simulink model "ModeStatAndRsp"  (R2018b)
settings: Solver=FixedStepDiscrete  StartTime=0.0  StopTime=10.0  FixedStep=0.01  RelTol=1e-3
undefined symbols (not defined in the file): c_RecvL, c_RecvLR, c_RecvR, IfVeSMSeStNumConfig, KeSMSbMdChime2Enable_Val, KeSMSbSRSPosNumConfig_Val, KeSMSuChmReqDurnTm_Val, KeSMSuChmReqIntlTm_Val, KeSMSuRspStatHldTm_Val, MdRspLocal1, MdTp1, ModeNum, PowerMode1, SrcReqTp1, srsconvert
libraries: RspLib x47, simulink x1
(part 1 of 8)
settings Model: ModifiedComment=sn2xws -- Mon May 30 15:02:40 2022 -- Version 1.7.1  Creator=Huanglu  LastModifiedBy=sn2xws
settings Model: ModifiedHistory=|
  | sn2xws -- Fri Dec 10 13:33:55 2021 -- Version 1.7.1
  | Vescom 7.0增加标定：KeSMSbMdChime2Enable
  | 
  | sn2xws -- Wed Oct 20 14:19:17 2021 -- Version 1.5.2
  | Bug 194428
  | StPassCmprtMd_RfCtrl_Sw_RclRspStat反馈增加新模式5个
  | sn2xws -- Wed Oct 20 14:19:17 2021 -- Version 1.5.1
  | bug 188541
  | 23.46数据库修改引起的增加模式5个
  | sn2xws -- Wed Oct 20 11:08:15 2021 -- Version 1.3.5
  | 4sbsy逻辑修改
  | 
  | sn2xws -- Thu Sep 23 09:51:03 2021 -- Version 1.3.4
  | 
  | sn2xws -- Thu Sep 23 09:16:20 2021 -- Version 1.3.4
  | 
  | sn2xws -- Thu Sep 23 08:52:00 2021 -- Version 1.3.4
  | 
  | sn2xws -- Wed Sep 22 16:44:24 2021 -- Version 1.3.4
  | 
  | sn2xws -- Wed Sep 22 16:34:35 2021 -- Version 1.3.4
  | 
  | sn2xws -- Mon Aug 30 09:30:48 2021 -- Version 1.3.4
  | 
  | sn2xws -- Mon Aug 30 09:23:49 2021 -- Version 1.3.4
  | IfVeSMSuSRSCrtMdIndTyp_67_2输出从0改为3
  | 
  | sn2xws -- Tue Aug 17 12:13:46 2021 -- Version 1.3.4
  | chime 的标定改为ms单位
  | 
  | sn2xws -- Thu Aug 12 14:48:49 2021 -- Version 1.3.3
  | CR147492 :
  | 退出时先看是否在位置，在位置则报成功，不报打断失败。
  | 
  | sn2xws -- Thu Aug 12 14:45:00 2021 -- Version 1.3.2
  | CR 147498 :模式当前状态反馈逻辑更新
  | Version 1.3.1
  | cr145167:修改chime逻辑并增加chime标定
settings DataIOCC: SaveFormat=StructureWithTime
settings OptimizationCC: DefaultParameterBehavior=Inlined  EnhancedBackFolding=on  PassReuseOutputArgsAs=Individual arguments  ZeroExternalMemoryAtStartup=off  ZeroInternalMemoryAtStartup=off  OptimizeBlockOrder=speed  DifferentSizesBufferReuse=on  OptimizationCustomize=off
settings DebuggingCC: ParameterTunabilityLossMsg=error  UnconnectedInputMsg=none  UnconnectedOutputMsg=none  UnconnectedLineMsg=none
settings ModelReferenceCC: ModelReferenceNumInstancesAllowed=Single
settings SFSimCC: MATLABDynamicMemAlloc=off
settings RTWCC: SystemTargetFile=autosar.tlc  GenCodeOnly=on  TemplateMakefile=ert_default_tmf  Description=AUTOSAR  GenerateReport=on  IncludeHyperlinkInReport=on  LaunchReport=on  GenerateTraceInfo=on  GenerateTraceReport=on  GenerateTraceReportSl=on  GenerateTraceReportSf=on  GenerateTraceReportEml=on
settings CodeAppCC: ForceParamTrailComments=on  IgnoreCustomStorageClasses=off  OperatorAnnotations=on  SimulinkDataObjDesc=on  SFDataObjDesc=on  InsertBlockDesc=on
settings STFCustomTargetCC: TargetLangStandard=C99 (ISO)  MultiwordLength=256  ParMdlRefBuildCompliant=on  CompOptLevelCompliant=on  IncludeMdlTerminateFcn=off  CombineOutputUpdateFcns=on  SuppressErrorStatus=on  ERTCustomFileBanners=on  SupportNonFinite=off  SupportComplex=off  SupportContinuousTime=off  SupportNonInlinedSFcns=off  RemoveResetFunc=on  MATLABClassNameForMDSCustomization=Simulink.SoftwareTarget.ERTCustomization  AutosarCompliant=on  UseToolchainInfoCompliant=on  LookupTableObjectStructAxisOrder=2,1,3,4,...  LUTObjectStructOrderEvenSpacing=Size,Table,Breakpoints  SystemTargetFile=autosar.tlc
settings ERTTargetCC: TargetLangStandard=C99 (ISO)  ConcurrentExecutionCompliant=off  IncludeMdlTerminateFcn=off  SuppressErrorStatus=on  SupportNonFinite=off  SupportComplex=off  ModelStepFunctionPrototypeControlCompliant=off  CPPClassGenCompliant=off  AutosarCompliant=on  LookupTableObjectStructAxisOrder=2,1,3,4,...  LUTObjectStructOrderEvenSpacing=Size,Table,Breakpoints  InlinedParameterPlacement=NonHierarchical  ERTCustomFileTemplate=example_file_process.tlc

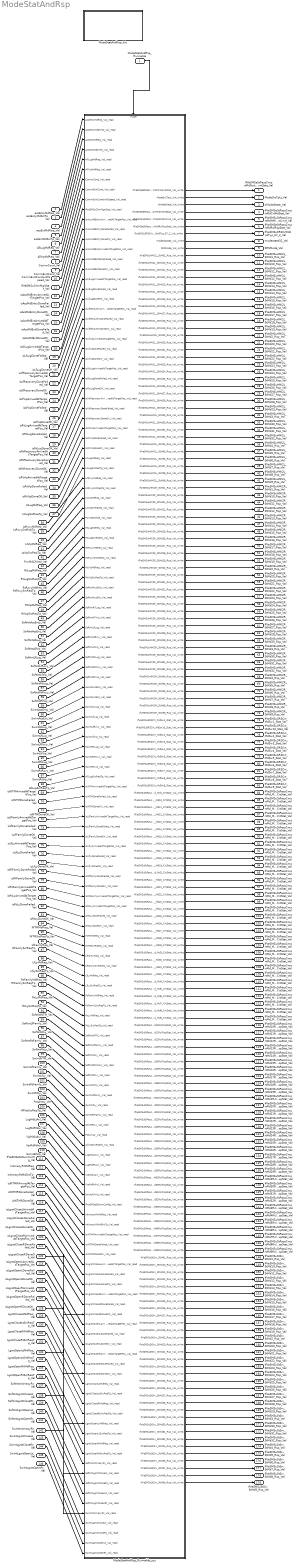
== system ModeStatAndRsp ==
  ModeStatAndRsp_Runnable : Inport  SampleTime=0.01  OutputFunctionCall=on
  acsEntyMdReq_Val : Inport  Port=2  OutDataTypeStr=boolean  PortDimensions=1
  acsEntyMdSrcTp_Val : Inport  Port=3  OutDataTypeStr=Enum: SrcReqTp1  PortDimensions=1
  acsExtMdReq_Val : Inport  Port=4  OutDataTypeStr=boolean  PortDimensions=1
  acsExtMdSrcTp_Val : Inport  Port=5  OutDataTypeStr=Enum: SrcReqTp1  PortDimensions=1
  AllLugMdReq_Val : Inport  Port=6  OutDataTypeStr=boolean  PortDimensions=1
  AllVipMdReq_Val : Inport  Port=7  OutDataTypeStr=boolean  PortDimensions=1
  CommCond_Val : Inport  Port=8  OutDataTypeStr=boolean  PortDimensions=1
  CommExitCond_Val : Inport  Port=9  OutDataTypeStr=boolean  PortDimensions=1
  CommExitCondwithSpeed_Val : Inport  Port=10  OutDataTypeStr=boolean  PortDimensions=1
  IfVeSMSuChmMgrStat_Val : Inport  Port=11  OutDataTypeStr=uint16  PortDimensions=1
  isAcsMdEntryArrivedAtTargetPos_Val : Inport  Port=12  OutDataTypeStr=boolean  PortDimensions=1
  isAcsMdEntryDoneFailed_Val : Inport  Port=13  OutDataTypeStr=boolean  PortDimensions=1
  isAcsMdEntryDoneOK_Val : Inport  Port=14  OutDataTypeStr=boolean  PortDimensions=1
  isAcsMdExtArrivedAtTargetPos_Val : Inport  Port=15  OutDataTypeStr=boolean  PortDimensions=1
  isAcsMdExtDoneFailed_Val : Inport  Port=16  OutDataTypeStr=boolean  PortDimensions=1
  isAcsMdExtDoneOK_Val : Inport  Port=17  OutDataTypeStr=boolean  PortDimensions=1
  isLfLugArrivedAtTargetPos_Val : Inport  Port=18  OutDataTypeStr=boolean  PortDimensions=1
  isLfLugDoneFailed_Val : Inport  Port=19  OutDataTypeStr=boolean  PortDimensions=1
  isLfLugDoneOK_Val : Inport  Port=20  OutDataTypeStr=boolean  PortDimensions=1
  isLfRecoveryArrivedAtTargetPos_Val : Inport  Port=21  OutDataTypeStr=boolean  PortDimensions=1
  isLfRecoveryDoneFailed_Val : Inport  Port=22  OutDataTypeStr=boolean  PortDimensions=1
  isLfRecoveryDoneOK_Val : Inport  Port=23  OutDataTypeStr=boolean  PortDimensions=1
  isLfVipArrivedAtTargetPos_Val : Inport  Port=24  OutDataTypeStr=boolean  PortDimensions=1
  isLfVipDoneFailed_Val : Inport  Port=25  OutDataTypeStr=boolean  PortDimensions=1
  isLfVipDoneOK_Val : Inport  Port=26  OutDataTypeStr=boolean  PortDimensions=1
  isRtLugArrivedAtTargetPos_Val : Inport  Port=27  OutDataTypeStr=boolean  PortDimensions=1
  isRtLugDoneFailed_Val : Inport  Port=28  OutDataTypeStr=boolean  PortDimensions=1
  isRtLugDoneOK_Val : Inport  Port=29  OutDataTypeStr=boolean  PortDimensions=1
  isRtRecoveryArrivedAtTargetPos_Val : Inport  Port=30  OutDataTypeStr=boolean  PortDimensions=1
  isRtRecoveryDoneFailed_Val : Inport  Port=31  OutDataTypeStr=boolean  PortDimensions=1
  isRtRecoveryDoneOK_Val : Inport  Port=32  OutDataTypeStr=boolean  PortDimensions=1
  isRtVipArrivedAtTargetPos_Val : Inport  Port=33  OutDataTypeStr=boolean  PortDimensions=1
  isRtVipDoneFailed_Val : Inport  Port=34  OutDataTypeStr=boolean  PortDimensions=1
  isRtVipDoneOK_Val : Inport  Port=35  OutDataTypeStr=boolean  PortDimensions=1
  LtLugMdReq_Val : Inport  Port=36  OutDataTypeStr=boolean  PortDimensions=1
  LtLugSrcReqTp_Val : Inport  Port=37  OutDataTypeStr=Enum: SrcReqTp1  PortDimensions=1
  LtRcvyMdReq_Val : Inport  Port=38  OutDataTypeStr=boolean  PortDimensions=1
  LtRcvySrcReqTp_Val : Inport  Port=39  OutDataTypeStr=Enum: SrcReqTp1  PortDimensions=1
  LtVipMdReq_Val : Inport  Port=40  OutDataTypeStr=boolean  PortDimensions=1
  LtVipSrcReqTp_Val : Inport  Port=41  OutDataTypeStr=Enum: SrcReqTp1  PortDimensions=1
  PwrMdChked_Val : Inport  Port=42  OutDataTypeStr=Enum: PowerMode1  PortDimensions=1
  RtLugMdReq_Val : Inport  Port=43  OutDataTypeStr=boolean  PortDimensions=1
  RtLugSrcReqTp_Val : Inport  Port=44  OutDataTypeStr=Enum: SrcReqTp1  PortDimensions=1
  RtRcvyMdReq_Val : Inport  Port=45  OutDataTypeStr=boolean  PortDimensions=1
  RtRcvySrcReqTp_Val : Inport  Port=46  OutDataTypeStr=Enum: SrcReqTp1  PortDimensions=1
  RtVipMdReq_Val : Inport  Port=47  OutDataTypeStr=boolean  PortDimensions=1
  RtVipSrcReqTp_Val : Inport  Port=48  OutDataTypeStr=Enum: SrcReqTp1  PortDimensions=1
  SoftIntAcsEnty_Val : Inport  Port=49  OutDataTypeStr=boolean  PortDimensions=1
  SoftIntAcsExt_Val : Inport  Port=50  OutDataTypeStr=boolean  PortDimensions=1
  SoftIntAllLug_Val : Inport  Port=51  OutDataTypeStr=boolean  PortDimensions=1
  SoftIntAllVip_Val : Inport  Port=52  OutDataTypeStr=boolean  PortDimensions=1
  SoftIntLfLug_Val : Inport  Port=53  OutDataTypeStr=boolean  PortDimensions=1
  SoftIntLfRcvy_Val : Inport  Port=54  OutDataTypeStr=boolean  PortDimensions=1
  SoftIntLfVip_Val : Inport  Port=55  OutDataTypeStr=boolean  PortDimensions=1
  SoftIntRtLug_Val : Inport  Port=56  OutDataTypeStr=boolean  PortDimensions=1
  SoftIntRtRcvy_Val : Inport  Port=57  OutDataTypeStr=boolean  PortDimensions=1
  SoftIntRtVip_Val : Inport  Port=58  OutDataTypeStr=boolean  PortDimensions=1
  SwIntAcsEnty_Val : Inport  Port=59  OutDataTypeStr=boolean  PortDimensions=1
  SwIntAcsExt_Val : Inport  Port=60  OutDataTypeStr=boolean  PortDimensions=1
  SwIntAllLug_Val : Inport  Port=61  OutDataTypeStr=boolean  PortDimensions=1
  SwIntLfLug_Val : Inport  Port=62  OutDataTypeStr=boolean  PortDimensions=1
  SwIntLfRcvy_Val : Inport  Port=63  OutDataTypeStr=boolean  PortDimensions=1
  SwIntLfVip_Val : Inport  Port=64  OutDataTypeStr=boolean  PortDimensions=1
  SwIntRtLug_Val : Inport  Port=65  OutDataTypeStr=boolean  PortDimensions=1
  SwIntRtRcvy_Val : Inport  Port=66  OutDataTypeStr=boolean  PortDimensions=1
  SwIntRtVip_Val : Inport  Port=67  OutDataTypeStr=boolean  PortDimensions=1
  AllLugSrcReqTp_Val : Inport  Port=68  OutDataTypeStr=Enum: SrcReqTp1  PortDimensions=1
  isINTMArrivedAtTargetPos_Val : Inport  Port=69  OutDataTypeStr=boolean  PortDimensions=1
  isINTMDoneFailed_Val : Inport  Port=70  OutDataTypeStr=boolean  PortDimensions=1
  isINTMDoneOK_Val : Inport  Port=71  OutDataTypeStr=boolean  PortDimensions=1
  isLfFamlyArrivedAtTargetPos_Val : Inport  Port=72  OutDataTypeStr=boolean  PortDimensions=1
  isLfFamlyDoneFailed_Val : Inport  Port=73  OutDataTypeStr=boolean  PortDimensions=1
  isLfFamlyDoneOK_Val : Inport  Port=74  OutDataTypeStr=boolean  PortDimensions=1
  isLfLyArrivedAtTargetPos_Val : Inport  Port=75  OutDataTypeStr=boolean  PortDimensions=1
  isLfLyDoneFailed_Val : Inport  Port=76  OutDataTypeStr=boolean  PortDimensions=1
  isLfLyDoneOK_Val : Inport  Port=77  OutDataTypeStr=boolean  PortDimensions=1
  isRfFamlyDoneFailed_Val : Inport  Port=78  OutDataTypeStr=boolean  PortDimensions=1
  isRfFamlyDoneOK_Val : Inport  Port=79  OutDataTypeStr=boolean  PortDimensions=1
  isRtFamlyArrivedAtTargetPos_Val : Inport  Port=80  OutDataTypeStr=boolean  PortDimensions=1
  isRtLyArrivedAtTargetPos_Val : Inport  Port=81  OutDataTypeStr=boolean  PortDimensions=1
  isRtLyDoneFailed_Val : Inport  Port=82  OutDataTypeStr=boolean  PortDimensions=1
  isRtLyDoneOK_Val : Inport  Port=83  OutDataTypeStr=boolean  PortDimensions=1
  INTMMdReq_Val : Inport  Port=84  OutDataTypeStr=boolean  PortDimensions=1
  INTMSrcReqTp_Val : Inport  Port=85  OutDataTypeStr=Enum: SrcReqTp1  PortDimensions=1
  LfFamlyReq_Val : Inport  Port=86  OutDataTypeStr=boolean  PortDimensions=1
  LfFamlySrcReqTp_Val : Inport  Port=87  OutDataTypeStr=Enum: SrcReqTp1  PortDimensions=1
  LfLyMdReq_Val : Inport  Port=88  OutDataTypeStr=boolean  PortDimensions=1
  LfLySrcReqTp_Val : Inport  Port=89  OutDataTypeStr=Enum: SrcReqTp1  PortDimensions=1
  RtFamlyMdReq_Val : Inport  Port=90  OutDataTypeStr=boolean  PortDimensions=1
  RtFamlySrcReqTp_Val : Inport  Port=91  OutDataTypeStr=Enum: SrcReqTp1  PortDimensions=1
  RtLyMdReq_Val : Inport  Port=92  OutDataTypeStr=boolean  PortDimensions=1
  RtLySrcReqTp_Val : Inport  Port=93  OutDataTypeStr=Enum: SrcReqTp1  PortDimensions=1
  SoftIntINTM_Val : Inport  Port=94  OutDataTypeStr=boolean  PortDimensions=1
  SoftIntLfFamly_Val : Inport  Port=95  OutDataTypeStr=boolean  PortDimensions=1
  SoftIntLfLy_Val : Inport  Port=96  OutDataTypeStr=boolean  PortDimensions=1
  SoftIntRtFamly_Val : Inport  Port=97  OutDataTypeStr=boolean  PortDimensions=1
  SoftIntRtLy_Val : Inport  Port=98  OutDataTypeStr=boolean  PortDimensions=1
  SwIntINTM_Val : Inport  Port=99  OutDataTypeStr=boolean  PortDimensions=1
  SwIntLfFamly_Val : Inport  Port=100  OutDataTypeStr=boolean  PortDimensions=1
  SwIntLfLy_Val : Inport  Port=101  OutDataTypeStr=boolean  PortDimensions=1
  SwIntRtFamly_Val : Inport  Port=102  OutDataTypeStr=boolean  PortDimensions=1
  SwIntRtLy_Val : Inport  Port=103  OutDataTypeStr=boolean  PortDimensions=1
  PosArray_Val : Inport  Port=104  OutDataTypeStr=uint8  PortDimensions=11
  AllVipSrcReqTp_Val : Inport  Port=105  OutDataTypeStr=Enum: SrcReqTp1  PortDimensions=1
  LugMdLtAvl_Val : Inport  Port=106  OutDataTypeStr=boolean  PortDimensions=1
  LugMdRtAvl_Val : Inport  Port=107  OutDataTypeStr=boolean  PortDimensions=1
  VipMdLtAvl_Val : Inport  Port=108  OutDataTypeStr=boolean  PortDimensions=1
  VipMdRtAvl_Val : Inport  Port=109  OutDataTypeStr=boolean  PortDimensions=1
  SwIntAllVip_Val : Inport  Port=110  OutDataTypeStr=IntEnable  PortDimensions=1
  IfVeSMSeStNumConfig_Val : Inport  Port=111  OutDataTypeStr=Enum: IfVeSMSeStNumConfig  PortDimensions=1
  IntimacyRtMdReq_Val : Inport  Port=112  OutDataTypeStr=boolean  PortDimensions=1
  IntimacyRtMdSrcTp_Val : Inport  Port=113  OutDataTypeStr=Enum: SrcReqTp1  PortDimensions=1
  isINTMRArrivedAtTargetPos_Val : Inport  Port=114  OutDataTypeStr=boolean  PortDimensions=1
  isINTMRDoneFailed_Val : Inport  Port=115  OutDataTypeStr=boolean  PortDimensions=1
  isINTMRDoneOK_Val : Inport  Port=116  OutDataTypeStr=boolean  PortDimensions=1
  isLgrstCloseLArrivedAtTargetPos_Val : Inport  Port=117  OutDataTypeStr=boolean  PortDimensions=1
  isLgrstCloseLDoneFailed_Val : Inport  Port=118  OutDataTypeStr=boolean  PortDimensions=1
  isLgrstCloseLDoneOK_Val : Inport  Port=119  OutDataTypeStr=boolean  PortDimensions=1
  isLgrstCloseRArrivedAtTargetPos_Val : Inport  Port=120  OutDataTypeStr=boolean  PortDimensions=1
  isLgrstCloseRDoneFailed_Val : Inport  Port=121  OutDataTypeStr=boolean  PortDimensions=1
  isLgrstCloseRDoneOK_Val : Inport  Port=122  OutDataTypeStr=boolean  PortDimensions=1
  isLgrstOpenLArrivedAtTargetPos_Val : Inport  Port=123  OutDataTypeStr=boolean  PortDimensions=1
  isLgrstOpenLDoneFailed_Val : Inport  Port=124  OutDataTypeStr=boolean  PortDimensions=1
  isLgrstOpenLDoneOK_Val : Inport  Port=125  OutDataTypeStr=boolean  PortDimensions=1
  isLgrstOpenRArrivedAtTargetPos_Val : Inport  Port=126  OutDataTypeStr=boolean  PortDimensions=1
  isLgrstOpenRDoneFailed_Val : Inport  Port=127  OutDataTypeStr=boolean  PortDimensions=1
  isLgrstOpenRDoneOK_Val : Inport  Port=128  OutDataTypeStr=boolean  PortDimensions=1
  LgrstCloseLtMdReq_Val : Inport  Port=129  OutDataTypeStr=boolean  PortDimensions=1
  LgrstCloseLtSrcReqTp_Val : Inport  Port=130  OutDataTypeStr=Enum: SrcReqTp1  PortDimensions=1
  LgrstCloseRtMdReq_Val : Inport  Port=131  OutDataTypeStr=boolean  PortDimensions=1
  LgrstCloseRtSrcReqTp_Val : Inport  Port=132  OutDataTypeStr=Enum: SrcReqTp1  PortDimensions=1
  LgrstOpenLtMdReq_Val : Inport  Port=133  OutDataTypeStr=boolean  PortDimensions=1
  LgrstOpenLtSrcReqTp_Val : Inport  Port=134  OutDataTypeStr=Enum: SrcReqTp1  PortDimensions=1
  LgrstOpenRtMdReq_Val : Inport  Port=135  OutDataTypeStr=boolean  PortDimensions=1
  LgrstOpenRtSrcReqTp_Val : Inport  Port=136  OutDataTypeStr=Enum: SrcReqTp1  PortDimensions=1
  SoftIntIntimacyRt_Val : Inport  Port=137  OutDataTypeStr=IntEnable  PortDimensions=1
  SoftIntLgrstCloseLt_Val : Inport  Port=138  OutDataTypeStr=IntEnable  PortDimensions=1
  SoftIntLgrstCloseRt_Val : Inport  Port=139  OutDataTypeStr=IntEnable  PortDimensions=1
  SoftIntLgrstOpenLt_Val : Inport  Port=140  OutDataTypeStr=IntEnable  PortDimensions=1
  SoftIntLgrstOpenRt_Val : Inport  Port=141  OutDataTypeStr=IntEnable  PortDimensions=1
  SwIntIntimacyRt_Val : Inport  Port=142  OutDataTypeStr=IntEnable  PortDimensions=1
  SwIntLgrstCloseLt_Val : Inport  Port=143  OutDataTypeStr=IntEnable  PortDimensions=1
  SwIntLgrstCloseRt_Val : Inport  Port=144  OutDataTypeStr=IntEnable  PortDimensions=1
  SwIntLgrstOpenLt_Val : Inport  Port=145  OutDataTypeStr=IntEnable  PortDimensions=1
  SwIntLgrstOpenRt_Val : Inport  Port=146  OutDataTypeStr=IntEnable  PortDimensions=1
  ModeStatAndRsp_Init : Subsystem
  ModeStatAndRsp_Runnable_sys : Subsystem
  IfVeSMSeStPassCmprtMdNoti2ChmEvntStat_Val : Outport  OutDataTypeStr=Enum: EventSts1  PortDimensions=1
  ModeSrcTpLt_Val : Outport  Port=2  OutDataTypeStr=Enum: SrcReqTp1  PortDimensions=1
  oModeState_Val : Outport  Port=3  OutDataTypeStr=Enum: MdTp1  PortDimensions=1
  IfVeSMSeStPassCmprtMdCrtMdStat_Val : Outport  Port=4  OutDataTypeStr=uint8  PortDimensions=1
  IfVeSMSuStPassCmprtMdHMIDisCmd_Val : Outport  Port=5  OutDataTypeStr=uint8  PortDimensions=1
  IfVeSMSeStPassCmprtMdRclRspStat_Val : Outport  Port=6  OutDataTypeStr=uint8  PortDimensions=1
  IfVeSMSuSRSCrtMdIndTyp_67_2_Val : Outport  Port=7  OutDataTypeStr=uint8  PortDimensions=1
  modestate32_Val : Outport  Port=8  OutDataTypeStr=uint32  PortDimensions=1
  SRSMode_Val : Outport  Port=9  OutDataTypeStr=Enum: SRSCurMode1  PortDimensions=1
  IfVeSMSuHMI2L_StMd1_Rsp_Val : Outport  Port=10  OutDataTypeStr=uint8  PortDimensions=1
  IfVeSMSuHMI2L_StMd10_Rsp_Val : Outport  Port=11  OutDataTypeStr=uint8  PortDimensions=1
  IfVeSMSuHMI2L_StMd11_Rsp_Val : Outport  Port=12  OutDataTypeStr=uint8  PortDimensions=1
  IfVeSMSuHMI2L_StMd12_Rsp_Val : Outport  Port=13  OutDataTypeStr=uint8  PortDimensions=1
  IfVeSMSuHMI2L_StMd13_Rsp_Val : Outport  Port=14  OutDataTypeStr=uint8  PortDimensions=1
  IfVeSMSuHMI2L_StMd14_Rsp_Val : Outport  Port=15  OutDataTypeStr=uint8  PortDimensions=1
  IfVeSMSuHMI2L_StMd15_Rsp_Val : Outport  Port=16  OutDataTypeStr=uint8  PortDimensions=1
  IfVeSMSuHMI2L_StMd16_Rsp_Val : Outport  Port=17  OutDataTypeStr=uint8  PortDimensions=1
  IfVeSMSuHMI2L_StMd17_Rsp_Val : Outport  Port=18  OutDataTypeStr=uint8  PortDimensions=1
  IfVeSMSuHMI2L_StMd18_Rsp_Val : Outport  Port=19  OutDataTypeStr=uint8  PortDimensions=1
  IfVeSMSuHMI2L_StMd19_Rsp_Val : Outport  Port=20  OutDataTypeStr=uint8  PortDimensions=1
  IfVeSMSuHMI2L_StMd2_Rsp_Val : Outport  Port=21  OutDataTypeStr=uint8  PortDimensions=1
  IfVeSMSuHMI2L_StMd20_Rsp_Val : Outport  Port=22  OutDataTypeStr=uint8  PortDimensions=1
  IfVeSMSuHMI2L_StMd21_Rsp_Val : Outport  Port=23  OutDataTypeStr=uint8  PortDimensions=1
  IfVeSMSuHMI2L_StMd22_Rsp_Val : Outport  Port=24  OutDataTypeStr=uint8  PortDimensions=1
  IfVeSMSuHMI2L_StMd23_Rsp_Val : Outport  Port=25  OutDataTypeStr=uint8  PortDimensions=1
  IfVeSMSuHMI2L_StMd24_Rsp_Val : Outport  Port=26  OutDataTypeStr=uint8  PortDimensions=1
  IfVeSMSuHMI2L_StMd25_Rsp_Val : Outport  Port=27  OutDataTypeStr=uint8  PortDimensions=1
  IfVeSMSuHMI2L_StMd26_Rsp_Val : Outport  Port=28  OutDataTypeStr=uint8  PortDimensions=1
  IfVeSMSuHMI2L_StMd27_Rsp_Val : Outport  Port=29  OutDataTypeStr=uint8  PortDimensions=1
  IfVeSMSuHMI2L_StMd28_Rsp_Val : Outport  Port=30  OutDataTypeStr=uint8  PortDimensions=1
  IfVeSMSuHMI2L_StMd29_Rsp_Val : Outport  Port=31  OutDataTypeStr=uint8  PortDimensions=1
  IfVeSMSuHMI2L_StMd3_Rsp_Val : Outport  Port=32  OutDataTypeStr=uint8  PortDimensions=1
  IfVeSMSuHMI2L_StMd30_Rsp_Val : Outport  Port=33  OutDataTypeStr=uint8  PortDimensions=1
  IfVeSMSuHMI2L_StMd31_Rsp_Val : Outport  Port=34  OutDataTypeStr=uint8  PortDimensions=1
  IfVeSMSuHMI2L_StMd32_Rsp_Val : Outport  Port=35  OutDataTypeStr=uint8  PortDimensions=1
  IfVeSMSuHMI2L_StMd4_Rsp_Val : Outport  Port=36  OutDataTypeStr=uint8  PortDimensions=1
  IfVeSMSuHMI2L_StMd5_Rsp_Val : Outport  Port=37  OutDataTypeStr=uint8  PortDimensions=1
  IfVeSMSuHMI2L_StMd6_Rsp_Val : Outport  Port=38  OutDataTypeStr=uint8  PortDimensions=1
  IfVeSMSuHMI2L_StMd7_Rsp_Val : Outport  Port=39  OutDataTypeStr=uint8  PortDimensions=1
  IfVeSMSuHMI2L_StMd8_Rsp_Val : Outport  Port=40  OutDataTypeStr=uint8  PortDimensions=1
  IfVeSMSuHMI2L_StMd9_Rsp_Val : Outport  Port=41  OutDataTypeStr=uint8  PortDimensions=1
  IfVeSMSuHMI2R_StMd1_Rsp_Val : Outport  Port=42  OutDataTypeStr=uint8  PortDimensions=1
  IfVeSMSuHMI2R_StMd10_Rsp_Val : Outport  Port=43  OutDataTypeStr=uint8  PortDimensions=1
  IfVeSMSuHMI2R_StMd11_Rsp_Val : Outport  Port=44  OutDataTypeStr=uint8  PortDimensions=1
  IfVeSMSuHMI2R_StMd12_Rsp_Val : Outport  Port=45  OutDataTypeStr=uint8  PortDimensions=1
  IfVeSMSuHMI2R_StMd13_Rsp_Val : Outport  Port=46  OutDataTypeStr=uint8  PortDimensions=1
  IfVeSMSuHMI2R_StMd14_Rsp_Val : Outport  Port=47  OutDataTypeStr=uint8  PortDimensions=1
  IfVeSMSuHMI2R_StMd15_Rsp_Val : Outport  Port=48  OutDataTypeStr=uint8  PortDimensions=1
  IfVeSMSuHMI2R_StMd16_Rsp_Val : Outport  Port=49  OutDataTypeStr=uint8  PortDimensions=1
  IfVeSMSuHMI2R_StMd17_Rsp_Val : Outport  Port=50  OutDataTypeStr=uint8  PortDimensions=1
  IfVeSMSuHMI2R_StMd18_Rsp_Val : Outport  Port=51  OutDataTypeStr=uint8  PortDimensions=1
  IfVeSMSuHMI2R_StMd19_Rsp_Val : Outport  Port=52  OutDataTypeStr=uint8  PortDimensions=1
  IfVeSMSuHMI2R_StMd2_Rsp_Val : Outport  Port=53  OutDataTypeStr=uint8  PortDimensions=1
  IfVeSMSuHMI2R_StMd20_Rsp_Val : Outport  Port=54  OutDataTypeStr=uint8  PortDimensions=1
  IfVeSMSuHMI2R_StMd21_Rsp_Val : Outport  Port=55  OutDataTypeStr=uint8  PortDimensions=1
  IfVeSMSuHMI2R_StMd22_Rsp_Val : Outport  Port=56  OutDataTypeStr=uint8  PortDimensions=1
  IfVeSMSuHMI2R_StMd23_Rsp_Val : Outport  Port=57  OutDataTypeStr=uint8  PortDimensions=1
  IfVeSMSuHMI2R_StMd24_Rsp_Val : Outport  Port=58  OutDataTypeStr=uint8  PortDimensions=1
  IfVeSMSuHMI2R_StMd25_Rsp_Val : Outport  Port=59  OutDataTypeStr=uint8  PortDimensions=1
  IfVeSMSuHMI2R_StMd26_Rsp_Val : Outport  Port=60  OutDataTypeStr=uint8  PortDimensions=1
  IfVeSMSuHMI2R_StMd27_Rsp_Val : Outport  Port=61  OutDataTypeStr=uint8  PortDimensions=1
  IfVeSMSuHMI2R_StMd28_Rsp_Val : Outport  Port=62  OutDataTypeStr=uint8  PortDimensions=1
  IfVeSMSuHMI2R_StMd29_Rsp_Val : Outport  Port=63  OutDataTypeStr=uint8  PortDimensions=1
  IfVeSMSuHMI2R_StMd3_Rsp_Val : Outport  Port=64  OutDataTypeStr=uint8  PortDimensions=1
  IfVeSMSuHMI2R_StMd30_Rsp_Val : Outport  Port=65  OutDataTypeStr=uint8  PortDimensions=1
  IfVeSMSuHMI2R_StMd31_Rsp_Val : Outport  Port=66  OutDataTypeStr=uint8  PortDimensions=1
  IfVeSMSuHMI2R_StMd32_Rsp_Val : Outport  Port=67  OutDataTypeStr=uint8  PortDimensions=1
  IfVeSMSuHMI2R_StMd4_Rsp_Val : Outport  Port=68  OutDataTypeStr=uint8  PortDimensions=1
  IfVeSMSuHMI2R_StMd5_Rsp_Val : Outport  Port=69  OutDataTypeStr=uint8  PortDimensions=1
  IfVeSMSuHMI2R_StMd6_Rsp_Val : Outport  Port=70  OutDataTypeStr=uint8  PortDimensions=1
  IfVeSMSuHMI2R_StMd7_Rsp_Val : Outport  Port=71  OutDataTypeStr=uint8  PortDimensions=1
  IfVeSMSuHMI2R_StMd8_Rsp_Val : Outport  Port=72  OutDataTypeStr=uint8  PortDimensions=1
  IfVeSMSuHMI2R_StMd9_Rsp_Val : Outport  Port=73  OutDataTypeStr=uint8  PortDimensions=1
  IfVeSMSuSRSCrt_MdSw1_Stat_Val : Outport  Port=74  OutDataTypeStr=uint8  PortDimensions=1
  IfVeSMSuSRSCrt_MdSw10_Stat_Val : Outport  Port=75  OutDataTypeStr=uint8  PortDimensions=1
  IfVeSMSuSRSCrt_MdSw2_Stat_Val : Outport  Port=76  OutDataTypeStr=uint8  PortDimensions=1
  IfVeSMSuSRSCrt_MdSw3_Stat_Val : Outport  Port=77  OutDataTypeStr=uint8  PortDimensions=1
  IfVeSMSuSRSCrt_MdSw4_Stat_Val : Outport  Port=78  OutDataTypeStr=uint8  PortDimensions=1
  IfVeSMSuSRSCrt_MdSw5_Stat_Val : Outport  Port=79  OutDataTypeStr=uint8  PortDimensions=1
  IfVeSMSuSRSCrt_MdSw6_Stat_Val : Outport  Port=80  OutDataTypeStr=uint8  PortDimensions=1
  IfVeSMSuSRSCrt_MdSw7_Stat_Val : Outport  Port=81  OutDataTypeStr=uint8  PortDimensions=1
  IfVeSMSuSRSCrt_MdSw8_Stat_Val : Outport  Port=82  OutDataTypeStr=uint8  PortDimensions=1
  IfVeSMSuSRSCrt_MdSw9_Stat_Val : Outport  Port=83  OutDataTypeStr=uint8  PortDimensions=1
  IfVeSMSuStPassCmprtMd_Md1_CrtStat_Val : Outport  Port=84  OutDataTypeStr=uint8  PortDimensions=1
  IfVeSMSuStPassCmprtMd_Md10_CrtStat_Val : Outport  Port=85  OutDataTypeStr=uint8  PortDimensions=1
  IfVeSMSuStPassCmprtMd_Md11_CrtStat_Val : Outport  Port=86  OutDataTypeStr=uint8  PortDimensions=1
  IfVeSMSuStPassCmprtMd_Md12_CrtStat_Val : Outport  Port=87  OutDataTypeStr=uint8  PortDimensions=1
  IfVeSMSuStPassCmprtMd_Md13_CrtStat_Val : Outport  Port=88  OutDataTypeStr=uint8  PortDimensions=1
  IfVeSMSuStPassCmprtMd_Md14_CrtStat_Val : Outport  Port=89  OutDataTypeStr=uint8  PortDimensions=1
  IfVeSMSuStPassCmprtMd_Md15_CrtStat_Val : Outport  Port=90  OutDataTypeStr=uint8  PortDimensions=1
  IfVeSMSuStPassCmprtMd_Md16_CrtStat_Val : Outport  Port=91  OutDataTypeStr=uint8  PortDimensions=1
  IfVeSMSuStPassCmprtMd_Md17_CrtStat_Val : Outport  Port=92  OutDataTypeStr=uint8  PortDimensions=1
  IfVeSMSuStPassCmprtMd_Md18_CrtStat_Val : Outport  Port=93  OutDataTypeStr=uint8  PortDimensions=1
  IfVeSMSuStPassCmprtMd_Md19_CrtStat_Val : Outport  Port=94  OutDataTypeStr=uint8  PortDimensions=1
  IfVeSMSuStPassCmprtMd_Md2_CrtStat_Val : Outport  Port=95  OutDataTypeStr=uint8  PortDimensions=1
  IfVeSMSuStPassCmprtMd_Md20_CrtStat_Val : Outport  Port=96  OutDataTypeStr=uint8  PortDimensions=1
  IfVeSMSuStPassCmprtMd_Md21_CrtStat_Val : Outport  Port=97  OutDataTypeStr=uint8  PortDimensions=1
  IfVeSMSuStPassCmprtMd_Md22_CrtStat_Val : Outport  Port=98  OutDataTypeStr=uint8  PortDimensions=1
  IfVeSMSuStPassCmprtMd_Md23_CrtStat_Val : Outport  Port=99  OutDataTypeStr=uint8  PortDimensions=1
  IfVeSMSuStPassCmprtMd_Md24_CrtStat_Val : Outport  Port=100  OutDataTypeStr=uint8  PortDimensions=1
  IfVeSMSuStPassCmprtMd_Md25_CrtStat_Val : Outport  Port=101  OutDataTypeStr=uint8  PortDimensions=1
  IfVeSMSuStPassCmprtMd_Md26_CrtStat_Val : Outport  Port=102  OutDataTypeStr=uint8  PortDimensions=1
  IfVeSMSuStPassCmprtMd_Md27_CrtStat_Val : Outport  Port=103  OutDataTypeStr=uint8  PortDimensions=1
  IfVeSMSuStPassCmprtMd_Md28_CrtStat_Val : Outport  Port=104  OutDataTypeStr=uint8  PortDimensions=1
  IfVeSMSuStPassCmprtMd_Md29_CrtStat_Val : Outport  Port=105  OutDataTypeStr=uint8  PortDimensions=1
  IfVeSMSuStPassCmprtMd_Md3_CrtStat_Val : Outport  Port=106  OutDataTypeStr=uint8  PortDimensions=1
  IfVeSMSuStPassCmprtMd_Md30_CrtStat_Val : Outport  Port=107  OutDataTypeStr=uint8  PortDimensions=1
  IfVeSMSuStPassCmprtMd_Md31_CrtStat_Val : Outport  Port=108  OutDataTypeStr=uint8  PortDimensions=1
  IfVeSMSuStPassCmprtMd_Md32_CrtStat_Val : Outport  Port=109  OutDataTypeStr=uint8  PortDimensions=1
  IfVeSMSuStPassCmprtMd_Md4_CrtStat_Val : Outport  Port=110  OutDataTypeStr=uint8  PortDimensions=1
  IfVeSMSuStPassCmprtMd_Md5_CrtStat_Val : Outport  Port=111  OutDataTypeStr=uint8  PortDimensions=1
  IfVeSMSuStPassCmprtMd_Md6_CrtStat_Val : Outport  Port=112  OutDataTypeStr=uint8  PortDimensions=1
  IfVeSMSuStPassCmprtMd_Md7_CrtStat_Val : Outport  Port=113  OutDataTypeStr=uint8  PortDimensions=1
  IfVeSMSuStPassCmprtMd_Md8_CrtStat_Val : Outport  Port=114  OutDataTypeStr=uint8  PortDimensions=1
  IfVeSMSuStPassCmprtMd_Md9_CrtStat_Val : Outport  Port=115  OutDataTypeStr=uint8  PortDimensions=1
  IfVeSMSuStPassCmprtMd10RclRspStat_Val : Outport  Port=116  OutDataTypeStr=uint8  PortDimensions=1
  IfVeSMSuStPassCmprtMd11RclRspStat_Val : Outport  Port=117  OutDataTypeStr=uint8  PortDimensions=1
  IfVeSMSuStPassCmprtMd12RclRspStat_Val : Outport  Port=118  OutDataTypeStr=uint8  PortDimensions=1
  IfVeSMSuStPassCmprtMd13RclRspStat_Val : Outport  Port=119  OutDataTypeStr=uint8  PortDimensions=1
  IfVeSMSuStPassCmprtMd14RclRspStat_Val : Outport  Port=120  OutDataTypeStr=uint8  PortDimensions=1
  IfVeSMSuStPassCmprtMd15RclRspStat_Val : Outport  Port=121  OutDataTypeStr=uint8  PortDimensions=1
  IfVeSMSuStPassCmprtMd16RclRspStat_Val : Outport  Port=122  OutDataTypeStr=uint8  PortDimensions=1
  IfVeSMSuStPassCmprtMd17RclRspStat_Val : Outport  Port=123  OutDataTypeStr=uint8  PortDimensions=1
  IfVeSMSuStPassCmprtMd18RclRspStat_Val : Outport  Port=124  OutDataTypeStr=uint8  PortDimensions=1
  IfVeSMSuStPassCmprtMd19RclRspStat_Val : Outport  Port=125  OutDataTypeStr=uint8  PortDimensions=1
  IfVeSMSuStPassCmprtMd1RclRspStat_Val : Outport  Port=126  OutDataTypeStr=uint8  PortDimensions=1
  IfVeSMSuStPassCmprtMd20RclRspStat_Val : Outport  Port=127  OutDataTypeStr=uint8  PortDimensions=1
  IfVeSMSuStPassCmprtMd21RclRspStat_Val : Outport  Port=128  OutDataTypeStr=uint8  PortDimensions=1
  IfVeSMSuStPassCmprtMd22RclRspStat_Val : Outport  Port=129  OutDataTypeStr=uint8  PortDimensions=1
  IfVeSMSuStPassCmprtMd23RclRspStat_Val : Outport  Port=130  OutDataTypeStr=uint8  PortDimensions=1
  IfVeSMSuStPassCmprtMd24RclRspStat_Val : Outport  Port=131  OutDataTypeStr=uint8  PortDimensions=1
  IfVeSMSuStPassCmprtMd25RclRspStat_Val : Outport  Port=132  OutDataTypeStr=uint8  PortDimensions=1
  IfVeSMSuStPassCmprtMd26RclRspStat_Val : Outport  Port=133  OutDataTypeStr=uint8  PortDimensions=1
  IfVeSMSuStPassCmprtMd27RclRspStat_Val : Outport  Port=134  OutDataTypeStr=uint8  PortDimensions=1
  IfVeSMSuStPassCmprtMd28RclRspStat_Val : Outport  Port=135  OutDataTypeStr=uint8  PortDimensions=1
  IfVeSMSuStPassCmprtMd29RclRspStat_Val : Outport  Port=136  OutDataTypeStr=uint8  PortDimensions=1
  IfVeSMSuStPassCmprtMd2RclRspStat_Val : Outport  Port=137  OutDataTypeStr=uint8  PortDimensions=1
  IfVeSMSuStPassCmprtMd30RclRspStat_Val : Outport  Port=138  OutDataTypeStr=uint8  PortDimensions=1
  IfVeSMSuStPassCmprtMd31RclRspStat_Val : Outport  Port=139  OutDataTypeStr=uint8  PortDimensions=1
  IfVeSMSuStPassCmprtMd32RclRspStat_Val : Outport  Port=140  OutDataTypeStr=uint8  PortDimensions=1
  IfVeSMSuStPassCmprtMd3RclRspStat_Val : Outport  Port=141  OutDataTypeStr=uint8  PortDimensions=1
  IfVeSMSuStPassCmprtMd4RclRspStat_Val : Outport  Port=142  OutDataTypeStr=uint8  PortDimensions=1
  IfVeSMSuStPassCmprtMd5RclRspStat_Val : Outport  Port=143  OutDataTypeStr=uint8  PortDimensions=1
  IfVeSMSuStPassCmprtMd6RclRspStat_Val : Outport  Port=144  OutDataTypeStr=uint8  PortDimensions=1
  IfVeSMSuStPassCmprtMd7RclRspStat_Val : Outport  Port=145  OutDataTypeStr=uint8  PortDimensions=1
  IfVeSMSuStPassCmprtMd8RclRspStat_Val : Outport  Port=146  OutDataTypeStr=uint8  PortDimensions=1
  IfVeSMSuStPassCmprtMd9RclRspStat_Val : Outport  Port=147  OutDataTypeStr=uint8  PortDimensions=1
  IfVeSMSuStSrv_StMd1_Rsp_Val : Outport  Port=148  OutDataTypeStr=uint8  PortDimensions=1
  IfVeSMSuStSrv_StMd10_Rsp_Val : Outport  Port=149  OutDataTypeStr=uint8  PortDimensions=1
  IfVeSMSuStSrv_StMd11_Rsp_Val : Outport  Port=150  OutDataTypeStr=uint8  PortDimensions=1
  IfVeSMSuStSrv_StMd12_Rsp_Val : Outport  Port=151  OutDataTypeStr=uint8  PortDimensions=1
  IfVeSMSuStSrv_StMd13_Rsp_Val : Outport  Port=152  OutDataTypeStr=uint8  PortDimensions=1
  IfVeSMSuStSrv_StMd14_Rsp_Val : Outport  Port=153  OutDataTypeStr=uint8  PortDimensions=1
  IfVeSMSuStSrv_StMd15_Rsp_Val : Outport  Port=154  OutDataTypeStr=uint8  PortDimensions=1
  IfVeSMSuStSrv_StMd16_Rsp_Val : Outport  Port=155  OutDataTypeStr=uint8  PortDimensions=1
  IfVeSMSuStSrv_StMd17_Rsp_Val : Outport  Port=156  OutDataTypeStr=uint8  PortDimensions=1
  IfVeSMSuStSrv_StMd18_Rsp_Val : Outport  Port=157  OutDataTypeStr=uint8  PortDimensions=1
  IfVeSMSuStSrv_StMd19_Rsp_Val : Outport  Port=158  OutDataTypeStr=uint8  PortDimensions=1
  IfVeSMSuStSrv_StMd2_Rsp_Val : Outport  Port=159  OutDataTypeStr=uint8  PortDimensions=1
  IfVeSMSuStSrv_StMd20_Rsp_Val : Outport  Port=160  OutDataTypeStr=uint8  PortDimensions=1
  IfVeSMSuStSrv_StMd21_Rsp_Val : Outport  Port=161  OutDataTypeStr=uint8  PortDimensions=1
  IfVeSMSuStSrv_StMd22_Rsp_Val : Outport  Port=162  OutDataTypeStr=uint8  PortDimensions=1
  IfVeSMSuStSrv_StMd23_Rsp_Val : Outport  Port=163  OutDataTypeStr=uint8  PortDimensions=1
  IfVeSMSuStSrv_StMd24_Rsp_Val : Outport  Port=164  OutDataTypeStr=uint8  PortDimensions=1
  IfVeSMSuStSrv_StMd25_Rsp_Val : Outport  Port=165  OutDataTypeStr=uint8  PortDimensions=1
  IfVeSMSuStSrv_StMd26_Rsp_Val : Outport  Port=166  OutDataTypeStr=uint8  PortDimensions=1
  IfVeSMSuStSrv_StMd27_Rsp_Val : Outport  Port=167  OutDataTypeStr=uint8  PortDimensions=1
  IfVeSMSuStSrv_StMd28_Rsp_Val : Outport  Port=168  OutDataTypeStr=uint8  PortDimensions=1
  IfVeSMSuStSrv_StMd29_Rsp_Val : Outport  Port=169  OutDataTypeStr=uint8  PortDimensions=1
  IfVeSMSuStSrv_StMd3_Rsp_Val : Outport  Port=170  OutDataTypeStr=uint8  PortDimensions=1
  IfVeSMSuStSrv_StMd30_Rsp_Val : Outport  Port=171  OutDataTypeStr=uint8  PortDimensions=1
  IfVeSMSuStSrv_StMd31_Rsp_Val : Outport  Port=172  OutDataTypeStr=uint8  PortDimensions=1
  IfVeSMSuStSrv_StMd32_Rsp_Val : Outport  Port=173  OutDataTypeStr=uint8  PortDimensions=1
  IfVeSMSuStSrv_StMd4_Rsp_Val : Outport  Port=174  OutDataTypeStr=uint8  PortDimensions=1
  IfVeSMSuStSrv_StMd5_Rsp_Val : Outport  Port=175  OutDataTypeStr=uint8  PortDimensions=1
  IfVeSMSuStSrv_StMd6_Rsp_Val : Outport  Port=176  OutDataTypeStr=uint8  PortDimensions=1
  IfVeSMSuStSrv_StMd7_Rsp_Val : Outport  Port=177  OutDataTypeStr=uint8  PortDimensions=1
  IfVeSMSuStSrv_StMd8_Rsp_Val : Outport  Port=178  OutDataTypeStr=uint8  PortDimensions=1
  IfVeSMSuStSrv_StMd9_Rsp_Val : Outport  Port=179  OutDataTypeStr=uint8  PortDimensions=1
  wires:
  acsEntyMdReq_Val/1 -> ModeStatAndRsp_Runnable_sys/1(acsEntyMdReq_Val_read)
  acsEntyMdSrcTp_Val/1 -> ModeStatAndRsp_Runnable_sys/2(acsEntyMdSrcTp_Val_read)
  acsExtMdReq_Val/1 -> ModeStatAndRsp_Runnable_sys/3(acsExtMdReq_Val_read)
  acsExtMdSrcTp_Val/1 -> ModeStatAndRsp_Runnable_sys/4(acsExtMdSrcTp_Val_read)
  AllLugMdReq_Val/1 -> ModeStatAndRsp_Runnable_sys/5(AllLugMdReq_Val_read)
  AllVipMdReq_Val/1 -> ModeStatAndRsp_Runnable_sys/6(AllVipMdReq_Val_read)
  CommCond_Val/1 -> ModeStatAndRsp_Runnable_sys/7(CommCond_Val_read)
  CommExitCond_Val/1 -> ModeStatAndRsp_Runnable_sys/8(CommExitCond_Val_read)
  CommExitCondwithSpeed_Val/1 -> ModeStatAndRsp_Runnable_sys/9(CommExitCondwithSpeed_Val_read)
  IfVeSMSuChmMgrStat_Val/1 -> ModeStatAndRsp_Runnable_sys/10(IfVeSMSuChmMgrStat_Val_read)
  isAcsMdEntryArrivedAtTargetPos_Val/1 -> ModeStatAndRsp_Runnable_sys/11(isAcsMdEntryArrivedAtTargetPos_Val_read)
  isAcsMdEntryDoneFailed_Val/1 -> ModeStatAndRsp_Runnable_sys/12(isAcsMdEntryDoneFailed_Val_read)
  isAcsMdEntryDoneOK_Val/1 -> ModeStatAndRsp_Runnable_sys/13(isAcsMdEntryDoneOK_Val_read)
  isAcsMdExtArrivedAtTargetPos_Val/1 -> ModeStatAndRsp_Runnable_sys/14(isAcsMdExtArrivedAtTargetPos_Val_read)
  isAcsMdExtDoneFailed_Val/1 -> ModeStatAndRsp_Runnable_sys/15(isAcsMdExtDoneFailed_Val_read)
  isAcsMdExtDoneOK_Val/1 -> ModeStatAndRsp_Runnable_sys/16(isAcsMdExtDoneOK_Val_read)
  isLfLugArrivedAtTargetPos_Val/1 -> ModeStatAndRsp_Runnable_sys/17(isLfLugArrivedAtTargetPos_Val_read)
  isLfLugDoneFailed_Val/1 -> ModeStatAndRsp_Runnable_sys/18(isLfLugDoneFailed_Val_read)
  isLfLugDoneOK_Val/1 -> ModeStatAndRsp_Runnable_sys/19(isLfLugDoneOK_Val_read)
  isLfRecoveryArrivedAtTargetPos_Val/1 -> ModeStatAndRsp_Runnable_sys/20(isLfRecoveryArrivedAtTargetPos_Val_read)
  isLfRecoveryDoneFailed_Val/1 -> ModeStatAndRsp_Runnable_sys/21(isLfRecoveryDoneFailed_Val_read)
  isLfRecoveryDoneOK_Val/1 -> ModeStatAndRsp_Runnable_sys/22(isLfRecoveryDoneOK_Val_read)
  isLfVipArrivedAtTargetPos_Val/1 -> ModeStatAndRsp_Runnable_sys/23(isLfVipArrivedAtTargetPos_Val_read)
  isLfVipDoneFailed_Val/1 -> ModeStatAndRsp_Runnable_sys/24(isLfVipDoneFailed_Val_read)
  isLfVipDoneOK_Val/1 -> ModeStatAndRsp_Runnable_sys/25(isLfVipDoneOK_Val_read)
  isRtLugArrivedAtTargetPos_Val/1 -> ModeStatAndRsp_Runnable_sys/26(isRtLugArrivedAtTargetPos_Val_read)
  isRtLugDoneFailed_Val/1 -> ModeStatAndRsp_Runnable_sys/27(isRtLugDoneFailed_Val_read)
  isRtLugDoneOK_Val/1 -> ModeStatAndRsp_Runnable_sys/28(isRtLugDoneOK_Val_read)
  isRtRecoveryArrivedAtTargetPos_Val/1 -> ModeStatAndRsp_Runnable_sys/29(isRtRecoveryArrivedAtTargetPos_Val_read)
  isRtRecoveryDoneFailed_Val/1 -> ModeStatAndRsp_Runnable_sys/30(isRtRecoveryDoneFailed_Val_read)
  isRtRecoveryDoneOK_Val/1 -> ModeStatAndRsp_Runnable_sys/31(isRtRecoveryDoneOK_Val_read)
  isRtVipArrivedAtTargetPos_Val/1 -> ModeStatAndRsp_Runnable_sys/32(isRtVipArrivedAtTargetPos_Val_read)
  isRtVipDoneFailed_Val/1 -> ModeStatAndRsp_Runnable_sys/33(isRtVipDoneFailed_Val_read)
  isRtVipDoneOK_Val/1 -> ModeStatAndRsp_Runnable_sys/34(isRtVipDoneOK_Val_read)
  LtLugMdReq_Val/1 -> ModeStatAndRsp_Runnable_sys/35(LtLugMdReq_Val_read)
  LtLugSrcReqTp_Val/1 -> ModeStatAndRsp_Runnable_sys/36(LtLugSrcReqTp_Val_read)
  LtRcvyMdReq_Val/1 -> ModeStatAndRsp_Runnable_sys/37(LtRcvyMdReq_Val_read)
  LtRcvySrcReqTp_Val/1 -> ModeStatAndRsp_Runnable_sys/38(LtRcvySrcReqTp_Val_read)
  LtVipMdReq_Val/1 -> ModeStatAndRsp_Runnable_sys/39(LtVipMdReq_Val_read)
  LtVipSrcReqTp_Val/1 -> ModeStatAndRsp_Runnable_sys/40(LtVipSrcReqTp_Val_read)
  PwrMdChked_Val/1 -> ModeStatAndRsp_Runnable_sys/41(PwrMdChked_Val_read)
  RtLugMdReq_Val/1 -> ModeStatAndRsp_Runnable_sys/42(RtLugMdReq_Val_read)
  RtLugSrcReqTp_Val/1 -> ModeStatAndRsp_Runnable_sys/43(RtLugSrcReqTp_Val_read)
  RtRcvyMdReq_Val/1 -> ModeStatAndRsp_Runnable_sys/44(RtRcvyMdReq_Val_read)
  RtRcvySrcReqTp_Val/1 -> ModeStatAndRsp_Runnable_sys/45(RtRcvySrcReqTp_Val_read)
  RtVipMdReq_Val/1 -> ModeStatAndRsp_Runnable_sys/46(RtVipMdReq_Val_read)
  RtVipSrcReqTp_Val/1 -> ModeStatAndRsp_Runnable_sys/47(RtVipSrcReqTp_Val_read)
  SoftIntAcsEnty_Val/1 -> ModeStatAndRsp_Runnable_sys/48(SoftIntAcsEnty_Val_read)
  SoftIntAcsExt_Val/1 -> ModeStatAndRsp_Runnable_sys/49(SoftIntAcsExt_Val_read)
  SoftIntAllLug_Val/1 -> ModeStatAndRsp_Runnable_sys/50(SoftIntAllLug_Val_read)
  SoftIntAllVip_Val/1 -> ModeStatAndRsp_Runnable_sys/51(SoftIntAllVip_Val_read)
  SoftIntLfLug_Val/1 -> ModeStatAndRsp_Runnable_sys/52(SoftIntLfLug_Val_read)
  SoftIntLfRcvy_Val/1 -> ModeStatAndRsp_Runnable_sys/53(SoftIntLfRcvy_Val_read)
  SoftIntLfVip_Val/1 -> ModeStatAndRsp_Runnable_sys/54(SoftIntLfVip_Val_read)
  SoftIntRtLug_Val/1 -> ModeStatAndRsp_Runnable_sys/55(SoftIntRtLug_Val_read)
  SoftIntRtRcvy_Val/1 -> ModeStatAndRsp_Runnable_sys/56(SoftIntRtRcvy_Val_read)
  SoftIntRtVip_Val/1 -> ModeStatAndRsp_Runnable_sys/57(SoftIntRtVip_Val_read)
  SwIntAcsEnty_Val/1 -> ModeStatAndRsp_Runnable_sys/58(SwIntAcsEnty_Val_read)
  SwIntAcsExt_Val/1 -> ModeStatAndRsp_Runnable_sys/59(SwIntAcsExt_Val_read)
  SwIntAllLug_Val/1 -> ModeStatAndRsp_Runnable_sys/60(SwIntAllLug_Val_read)
  SwIntLfLug_Val/1 -> ModeStatAndRsp_Runnable_sys/61(SwIntLfLug_Val_read)
  SwIntLfRcvy_Val/1 -> ModeStatAndRsp_Runnable_sys/62(SwIntLfRcvy_Val_read)
  SwIntLfVip_Val/1 -> ModeStatAndRsp_Runnable_sys/63(SwIntLfVip_Val_read)
  SwIntRtLug_Val/1 -> ModeStatAndRsp_Runnable_sys/64(SwIntRtLug_Val_read)
  SwIntRtRcvy_Val/1 -> ModeStatAndRsp_Runnable_sys/65(SwIntRtRcvy_Val_read)
  SwIntRtVip_Val/1 -> ModeStatAndRsp_Runnable_sys/66(SwIntRtVip_Val_read)
  ModeStatAndRsp_Runnable_sys/1(IfVeSMSeStPassCmprtMdNoti2ChmEvntStat_Val_write) -> IfVeSMSeStPassCmprtMdNoti2ChmEvntStat_Val/1
  ModeStatAndRsp_Runnable_sys/2(ModeSrcTpLt_Val_write) -> ModeSrcTpLt_Val/1
  ModeStatAndRsp_Runnable_sys/3(oModeState_Val_write) -> oModeState_Val/1
  ModeStatAndRsp_Runnable_sys/4(IfVeSMSeStPassCmprtMdCrtMdStat_Val_write) -> IfVeSMSeStPassCmprtMdCrtMdStat_Val/1
  ModeStatAndRsp_Runnable_sys/5(IfVeSMSuStPassCmprtMdHMIDisCmd_Val_write) -> IfVeSMSuStPassCmprtMdHMIDisCmd_Val/1
  ModeStatAndRsp_Runnable_sys/6(IfVeSMSeStPassCmprtMdRclRspStat_Val_write) -> IfVeSMSeStPassCmprtMdRclRspStat_Val/1
  ModeStatAndRsp_Runnable/1 -> ModeStatAndRsp_Runnable_sys/Trigger
  AllLugSrcReqTp_Val/1 -> ModeStatAndRsp_Runnable_sys/67(AllLugSrcReqTp_Val_read)
  ModeStatAndRsp_Runnable_sys/7(IfVeSMSuSRSCrtMdIndTyp_67_2_Val_write) -> IfVeSMSuSRSCrtMdIndTyp_67_2_Val/1
  ModeStatAndRsp_Runnable_sys/8(modestate32_Val_write) -> modestate32_Val/1
  ModeStatAndRsp_Runnable_sys/9(SRSMode_Val_write) -> SRSMode_Val/1
  isINTMArrivedAtTargetPos_Val/1 -> ModeStatAndRsp_Runnable_sys/68(isINTMArrivedAtTargetPos_Val_read)
  isINTMDoneFailed_Val/1 -> ModeStatAndRsp_Runnable_sys/69(isINTMDoneFailed_Val_read)
  isINTMDoneOK_Val/1 -> ModeStatAndRsp_Runnable_sys/70(isINTMDoneOK_Val_read)
  isLfFamlyArrivedAtTargetPos_Val/1 -> ModeStatAndRsp_Runnable_sys/71(isLfFamlyArrivedAtTargetPos_Val_read)
  isLfFamlyDoneFailed_Val/1 -> ModeStatAndRsp_Runnable_sys/72(isLfFamlyDoneFailed_Val_read)
  isLfFamlyDoneOK_Val/1 -> ModeStatAndRsp_Runnable_sys/73(isLfFamlyDoneOK_Val_read)
  isLfLyArrivedAtTargetPos_Val/1 -> ModeStatAndRsp_Runnable_sys/74(isLfLyArrivedAtTargetPos_Val_read)
  isLfLyDoneFailed_Val/1 -> ModeStatAndRsp_Runnable_sys/75(isLfLyDoneFailed_Val_read)
  isLfLyDoneOK_Val/1 -> ModeStatAndRsp_Runnable_sys/76(isLfLyDoneOK_Val_read)
  isRfFamlyDoneFailed_Val/1 -> ModeStatAndRsp_Runnable_sys/77(isRfFamlyDoneFailed_Val_read)
  isRfFamlyDoneOK_Val/1 -> ModeStatAndRsp_Runnable_sys/78(isRfFamlyDoneOK_Val_read)
  isRtFamlyArrivedAtTargetPos_Val/1 -> ModeStatAndRsp_Runnable_sys/79(isRtFamlyArrivedAtTargetPos_Val_read)
  isRtLyArrivedAtTargetPos_Val/1 -> ModeStatAndRsp_Runnable_sys/80(isRtLyArrivedAtTargetPos_Val_read)
  isRtLyDoneFailed_Val/1 -> ModeStatAndRsp_Runnable_sys/81(isRtLyDoneFailed_Val_read)
  isRtLyDoneOK_Val/1 -> ModeStatAndRsp_Runnable_sys/82(isRtLyDoneOK_Val_read)
  ModeStatAndRsp_Runnable_sys/10(IfVeSMSuHMI2L_StMd1_Rsp_Val_write) -> IfVeSMSuHMI2L_StMd1_Rsp_Val/1
  ModeStatAndRsp_Runnable_sys/11(IfVeSMSuHMI2L_StMd10_Rsp_Val_write) -> IfVeSMSuHMI2L_StMd10_Rsp_Val/1
  ModeStatAndRsp_Runnable_sys/12(IfVeSMSuHMI2L_StMd11_Rsp_Val_write) -> IfVeSMSuHMI2L_StMd11_Rsp_Val/1
  ModeStatAndRsp_Runnable_sys/13(IfVeSMSuHMI2L_StMd12_Rsp_Val_write) -> IfVeSMSuHMI2L_StMd12_Rsp_Val/1
  ModeStatAndRsp_Runnable_sys/14(IfVeSMSuHMI2L_StMd13_Rsp_Val_write) -> IfVeSMSuHMI2L_StMd13_Rsp_Val/1
  ModeStatAndRsp_Runnable_sys/15(IfVeSMSuHMI2L_StMd14_Rsp_Val_write) -> IfVeSMSuHMI2L_StMd14_Rsp_Val/1
  ModeStatAndRsp_Runnable_sys/16(IfVeSMSuHMI2L_StMd15_Rsp_Val_write) -> IfVeSMSuHMI2L_StMd15_Rsp_Val/1
  ModeStatAndRsp_Runnable_sys/17(IfVeSMSuHMI2L_StMd16_Rsp_Val_write) -> IfVeSMSuHMI2L_StMd16_Rsp_Val/1
  ModeStatAndRsp_Runnable_sys/18(IfVeSMSuHMI2L_StMd17_Rsp_Val_write) -> IfVeSMSuHMI2L_StMd17_Rsp_Val/1
  ModeStatAndRsp_Runnable_sys/19(IfVeSMSuHMI2L_StMd18_Rsp_Val_write) -> IfVeSMSuHMI2L_StMd18_Rsp_Val/1
  ModeStatAndRsp_Runnable_sys/20(IfVeSMSuHMI2L_StMd19_Rsp_Val_write) -> IfVeSMSuHMI2L_StMd19_Rsp_Val/1
  ModeStatAndRsp_Runnable_sys/21(IfVeSMSuHMI2L_StMd2_Rsp_Val_write) -> IfVeSMSuHMI2L_StMd2_Rsp_Val/1
  ModeStatAndRsp_Runnable_sys/22(IfVeSMSuHMI2L_StMd20_Rsp_Val_write) -> IfVeSMSuHMI2L_StMd20_Rsp_Val/1
  ModeStatAndRsp_Runnable_sys/23(IfVeSMSuHMI2L_StMd21_Rsp_Val_write) -> IfVeSMSuHMI2L_StMd21_Rsp_Val/1
  ModeStatAndRsp_Runnable_sys/24(IfVeSMSuHMI2L_StMd22_Rsp_Val_write) -> IfVeSMSuHMI2L_StMd22_Rsp_Val/1
  ModeStatAndRsp_Runnable_sys/25(IfVeSMSuHMI2L_StMd23_Rsp_Val_write) -> IfVeSMSuHMI2L_StMd23_Rsp_Val/1
  ModeStatAndRsp_Runnable_sys/26(IfVeSMSuHMI2L_StMd24_Rsp_Val_write) -> IfVeSMSuHMI2L_StMd24_Rsp_Val/1
  ModeStatAndRsp_Runnable_sys/27(IfVeSMSuHMI2L_StMd25_Rsp_Val_write) -> IfVeSMSuHMI2L_StMd25_Rsp_Val/1
  ModeStatAndRsp_Runnable_sys/28(IfVeSMSuHMI2L_StMd26_Rsp_Val_write) -> IfVeSMSuHMI2L_StMd26_Rsp_Val/1
  ModeStatAndRsp_Runnable_sys/29(IfVeSMSuHMI2L_StMd27_Rsp_Val_write) -> IfVeSMSuHMI2L_StMd27_Rsp_Val/1
  ModeStatAndRsp_Runnable_sys/30(IfVeSMSuHMI2L_StMd28_Rsp_Val_write) -> IfVeSMSuHMI2L_StMd28_Rsp_Val/1
  ModeStatAndRsp_Runnable_sys/31(IfVeSMSuHMI2L_StMd29_Rsp_Val_write) -> IfVeSMSuHMI2L_StMd29_Rsp_Val/1
  ModeStatAndRsp_Runnable_sys/32(IfVeSMSuHMI2L_StMd3_Rsp_Val_write) -> IfVeSMSuHMI2L_StMd3_Rsp_Val/1
  ModeStatAndRsp_Runnable_sys/33(IfVeSMSuHMI2L_StMd30_Rsp_Val_write) -> IfVeSMSuHMI2L_StMd30_Rsp_Val/1
  ModeStatAndRsp_Runnable_sys/34(IfVeSMSuHMI2L_StMd31_Rsp_Val_write) -> IfVeSMSuHMI2L_StMd31_Rsp_Val/1
  ModeStatAndRsp_Runnable_sys/35(IfVeSMSuHMI2L_StMd32_Rsp_Val_write) -> IfVeSMSuHMI2L_StMd32_Rsp_Val/1
  ModeStatAndRsp_Runnable_sys/36(IfVeSMSuHMI2L_StMd4_Rsp_Val_write) -> IfVeSMSuHMI2L_StMd4_Rsp_Val/1
  ModeStatAndRsp_Runnable_sys/37(IfVeSMSuHMI2L_StMd5_Rsp_Val_write) -> IfVeSMSuHMI2L_StMd5_Rsp_Val/1
  ModeStatAndRsp_Runnable_sys/38(IfVeSMSuHMI2L_StMd6_Rsp_Val_write) -> IfVeSMSuHMI2L_StMd6_Rsp_Val/1
  ModeStatAndRsp_Runnable_sys/39(IfVeSMSuHMI2L_StMd7_Rsp_Val_write) -> IfVeSMSuHMI2L_StMd7_Rsp_Val/1
  ModeStatAndRsp_Runnable_sys/40(IfVeSMSuHMI2L_StMd8_Rsp_Val_write) -> IfVeSMSuHMI2L_StMd8_Rsp_Val/1
  ModeStatAndRsp_Runnable_sys/41(IfVeSMSuHMI2L_StMd9_Rsp_Val_write) -> IfVeSMSuHMI2L_StMd9_Rsp_Val/1
  ModeStatAndRsp_Runnable_sys/42(IfVeSMSuHMI2R_StMd1_Rsp_Val_write) -> IfVeSMSuHMI2R_StMd1_Rsp_Val/1
  ModeStatAndRsp_Runnable_sys/43(IfVeSMSuHMI2R_StMd10_Rsp_Val_write) -> IfVeSMSuHMI2R_StMd10_Rsp_Val/1
  ModeStatAndRsp_Runnable_sys/44(IfVeSMSuHMI2R_StMd11_Rsp_Val_write) -> IfVeSMSuHMI2R_StMd11_Rsp_Val/1
  ModeStatAndRsp_Runnable_sys/45(IfVeSMSuHMI2R_StMd12_Rsp_Val_write) -> IfVeSMSuHMI2R_StMd12_Rsp_Val/1
  ModeStatAndRsp_Runnable_sys/46(IfVeSMSuHMI2R_StMd13_Rsp_Val_write) -> IfVeSMSuHMI2R_StMd13_Rsp_Val/1
  ModeStatAndRsp_Runnable_sys/47(IfVeSMSuHMI2R_StMd14_Rsp_Val_write) -> IfVeSMSuHMI2R_StMd14_Rsp_Val/1
  ModeStatAndRsp_Runnable_sys/48(IfVeSMSuHMI2R_StMd15_Rsp_Val_write) -> IfVeSMSuHMI2R_StMd15_Rsp_Val/1
  ModeStatAndRsp_Runnable_sys/49(IfVeSMSuHMI2R_StMd16_Rsp_Val_write) -> IfVeSMSuHMI2R_StMd16_Rsp_Val/1
  ModeStatAndRsp_Runnable_sys/50(IfVeSMSuHMI2R_StMd17_Rsp_Val_write) -> IfVeSMSuHMI2R_StMd17_Rsp_Val/1
  ModeStatAndRsp_Runnable_sys/51(IfVeSMSuHMI2R_StMd18_Rsp_Val_write) -> IfVeSMSuHMI2R_StMd18_Rsp_Val/1
  ModeStatAndRsp_Runnable_sys/52(IfVeSMSuHMI2R_StMd19_Rsp_Val_write) -> IfVeSMSuHMI2R_StMd19_Rsp_Val/1
  ModeStatAndRsp_Runnable_sys/53(IfVeSMSuHMI2R_StMd2_Rsp_Val_write) -> IfVeSMSuHMI2R_StMd2_Rsp_Val/1
  ModeStatAndRsp_Runnable_sys/54(IfVeSMSuHMI2R_StMd20_Rsp_Val_write) -> IfVeSMSuHMI2R_StMd20_Rsp_Val/1
  ModeStatAndRsp_Runnable_sys/55(IfVeSMSuHMI2R_StMd21_Rsp_Val_write) -> IfVeSMSuHMI2R_StMd21_Rsp_Val/1
  ModeStatAndRsp_Runnable_sys/56(IfVeSMSuHMI2R_StMd22_Rsp_Val_write) -> IfVeSMSuHMI2R_StMd22_Rsp_Val/1
  ModeStatAndRsp_Runnable_sys/57(IfVeSMSuHMI2R_StMd23_Rsp_Val_write) -> IfVeSMSuHMI2R_StMd23_Rsp_Val/1
  ModeStatAndRsp_Runnable_sys/58(IfVeSMSuHMI2R_StMd24_Rsp_Val_write) -> IfVeSMSuHMI2R_StMd24_Rsp_Val/1
  ModeStatAndRsp_Runnable_sys/59(IfVeSMSuHMI2R_StMd25_Rsp_Val_write) -> IfVeSMSuHMI2R_StMd25_Rsp_Val/1
  ModeStatAndRsp_Runnable_sys/60(IfVeSMSuHMI2R_StMd26_Rsp_Val_write) -> IfVeSMSuHMI2R_StMd26_Rsp_Val/1
  ModeStatAndRsp_Runnable_sys/61(IfVeSMSuHMI2R_StMd27_Rsp_Val_write) -> IfVeSMSuHMI2R_StMd27_Rsp_Val/1
  ModeStatAndRsp_Runnable_sys/62(IfVeSMSuHMI2R_StMd28_Rsp_Val_write) -> IfVeSMSuHMI2R_StMd28_Rsp_Val/1
  ModeStatAndRsp_Runnable_sys/63(IfVeSMSuHMI2R_StMd29_Rsp_Val_write) -> IfVeSMSuHMI2R_StMd29_Rsp_Val/1
  ModeStatAndRsp_Runnable_sys/64(IfVeSMSuHMI2R_StMd3_Rsp_Val_write) -> IfVeSMSuHMI2R_StMd3_Rsp_Val/1
  ModeStatAndRsp_Runnable_sys/65(IfVeSMSuHMI2R_StMd30_Rsp_Val_write) -> IfVeSMSuHMI2R_StMd30_Rsp_Val/1
  ModeStatAndRsp_Runnable_sys/66(IfVeSMSuHMI2R_StMd31_Rsp_Val_write) -> IfVeSMSuHMI2R_StMd31_Rsp_Val/1
  ModeStatAndRsp_Runnable_sys/67(IfVeSMSuHMI2R_StMd32_Rsp_Val_write) -> IfVeSMSuHMI2R_StMd32_Rsp_Val/1
  ModeStatAndRsp_Runnable_sys/68(IfVeSMSuHMI2R_StMd4_Rsp_Val_write) -> IfVeSMSuHMI2R_StMd4_Rsp_Val/1
  ModeStatAndRsp_Runnable_sys/69(IfVeSMSuHMI2R_StMd5_Rsp_Val_write) -> IfVeSMSuHMI2R_StMd5_Rsp_Val/1
  ModeStatAndRsp_Runnable_sys/70(IfVeSMSuHMI2R_StMd6_Rsp_Val_write) -> IfVeSMSuHMI2R_StMd6_Rsp_Val/1
  ModeStatAndRsp_Runnable_sys/71(IfVeSMSuHMI2R_StMd7_Rsp_Val_write) -> IfVeSMSuHMI2R_StMd7_Rsp_Val/1
  ModeStatAndRsp_Runnable_sys/72(IfVeSMSuHMI2R_StMd8_Rsp_Val_write) -> IfVeSMSuHMI2R_StMd8_Rsp_Val/1
  ModeStatAndRsp_Runnable_sys/73(IfVeSMSuHMI2R_StMd9_Rsp_Val_write) -> IfVeSMSuHMI2R_StMd9_Rsp_Val/1
  ModeStatAndRsp_Runnable_sys/74(IfVeSMSuSRSCrt_MdSw1_Stat_Val_write) -> IfVeSMSuSRSCrt_MdSw1_Stat_Val/1
  ModeStatAndRsp_Runnable_sys/75(IfVeSMSuSRSCrt_MdSw10_Stat_Val_write) -> IfVeSMSuSRSCrt_MdSw10_Stat_Val/1
  ModeStatAndRsp_Runnable_sys/76(IfVeSMSuSRSCrt_MdSw2_Stat_Val_write) -> IfVeSMSuSRSCrt_MdSw2_Stat_Val/1
  ModeStatAndRsp_Runnable_sys/77(IfVeSMSuSRSCrt_MdSw3_Stat_Val_write) -> IfVeSMSuSRSCrt_MdSw3_Stat_Val/1
  ModeStatAndRsp_Runnable_sys/78(IfVeSMSuSRSCrt_MdSw4_Stat_Val_write) -> IfVeSMSuSRSCrt_MdSw4_Stat_Val/1
  ModeStatAndRsp_Runnable_sys/79(IfVeSMSuSRSCrt_MdSw5_Stat_Val_write) -> IfVeSMSuSRSCrt_MdSw5_Stat_Val/1
  ModeStatAndRsp_Runnable_sys/80(IfVeSMSuSRSCrt_MdSw6_Stat_Val_write) -> IfVeSMSuSRSCrt_MdSw6_Stat_Val/1
  ModeStatAndRsp_Runnable_sys/81(IfVeSMSuSRSCrt_MdSw7_Stat_Val_write) -> IfVeSMSuSRSCrt_MdSw7_Stat_Val/1
  ModeStatAndRsp_Runnable_sys/82(IfVeSMSuSRSCrt_MdSw8_Stat_Val_write) -> IfVeSMSuSRSCrt_MdSw8_Stat_Val/1
  ModeStatAndRsp_Runnable_sys/83(IfVeSMSuSRSCrt_MdSw9_Stat_Val_write) -> IfVeSMSuSRSCrt_MdSw9_Stat_Val/1
  ModeStatAndRsp_Runnable_sys/84(IfVeSMSuStPassCmprtMd_Md1_CrtStat_Val_write) -> IfVeSMSuStPassCmprtMd_Md1_CrtStat_Val/1
  ModeStatAndRsp_Runnable_sys/85(IfVeSMSuStPassCmprtMd_Md10_CrtStat_Val_write) -> IfVeSMSuStPassCmprtMd_Md10_CrtStat_Val/1
  ModeStatAndRsp_Runnable_sys/86(IfVeSMSuStPassCmprtMd_Md11_CrtStat_Val_write) -> IfVeSMSuStPassCmprtMd_Md11_CrtStat_Val/1
  ModeStatAndRsp_Runnable_sys/87(IfVeSMSuStPassCmprtMd_Md12_CrtStat_Val_write) -> IfVeSMSuStPassCmprtMd_Md12_CrtStat_Val/1
  ModeStatAndRsp_Runnable_sys/88(IfVeSMSuStPassCmprtMd_Md13_CrtStat_Val_write) -> IfVeSMSuStPassCmprtMd_Md13_CrtStat_Val/1
  ModeStatAndRsp_Runnable_sys/89(IfVeSMSuStPassCmprtMd_Md14_CrtStat_Val_write) -> IfVeSMSuStPassCmprtMd_Md14_CrtStat_Val/1
  ModeStatAndRsp_Runnable_sys/90(IfVeSMSuStPassCmprtMd_Md15_CrtStat_Val_write) -> IfVeSMSuStPassCmprtMd_Md15_CrtStat_Val/1
  ModeStatAndRsp_Runnable_sys/91(IfVeSMSuStPassCmprtMd_Md16_CrtStat_Val_write) -> IfVeSMSuStPassCmprtMd_Md16_CrtStat_Val/1
  ModeStatAndRsp_Runnable_sys/92(IfVeSMSuStPassCmprtMd_Md17_CrtStat_Val_write) -> IfVeSMSuStPassCmprtMd_Md17_CrtStat_Val/1
  ModeStatAndRsp_Runnable_sys/93(IfVeSMSuStPassCmprtMd_Md18_CrtStat_Val_write) -> IfVeSMSuStPassCmprtMd_Md18_CrtStat_Val/1
  ModeStatAndRsp_Runnable_sys/94(IfVeSMSuStPassCmprtMd_Md19_CrtStat_Val_write) -> IfVeSMSuStPassCmprtMd_Md19_CrtStat_Val/1
  ModeStatAndRsp_Runnable_sys/95(IfVeSMSuStPassCmprtMd_Md2_CrtStat_Val_write) -> IfVeSMSuStPassCmprtMd_Md2_CrtStat_Val/1
  ModeStatAndRsp_Runnable_sys/96(IfVeSMSuStPassCmprtMd_Md20_CrtStat_Val_write) -> IfVeSMSuStPassCmprtMd_Md20_CrtStat_Val/1
  ModeStatAndRsp_Runnable_sys/97(IfVeSMSuStPassCmprtMd_Md21_CrtStat_Val_write) -> IfVeSMSuStPassCmprtMd_Md21_CrtStat_Val/1
  ModeStatAndRsp_Runnable_sys/98(IfVeSMSuStPassCmprtMd_Md22_CrtStat_Val_write) -> IfVeSMSuStPassCmprtMd_Md22_CrtStat_Val/1
  ModeStatAndRsp_Runnable_sys/99(IfVeSMSuStPassCmprtMd_Md23_CrtStat_Val_write) -> IfVeSMSuStPassCmprtMd_Md23_CrtStat_Val/1
  ModeStatAndRsp_Runnable_sys/100(IfVeSMSuStPassCmprtMd_Md24_CrtStat_Val_write) -> IfVeSMSuStPassCmprtMd_Md24_CrtStat_Val/1
  ModeStatAndRsp_Runnable_sys/101(IfVeSMSuStPassCmprtMd_Md25_CrtStat_Val_write) -> IfVeSMSuStPassCmprtMd_Md25_CrtStat_Val/1
  ModeStatAndRsp_Runnable_sys/102(IfVeSMSuStPassCmprtMd_Md26_CrtStat_Val_write) -> IfVeSMSuStPassCmprtMd_Md26_CrtStat_Val/1
  ModeStatAndRsp_Runnable_sys/103(IfVeSMSuStPassCmprtMd_Md27_CrtStat_Val_write) -> IfVeSMSuStPassCmprtMd_Md27_CrtStat_Val/1
  ModeStatAndRsp_Runnable_sys/104(IfVeSMSuStPassCmprtMd_Md28_CrtStat_Val_write) -> IfVeSMSuStPassCmprtMd_Md28_CrtStat_Val/1
  ModeStatAndRsp_Runnable_sys/105(IfVeSMSuStPassCmprtMd_Md29_CrtStat_Val_write) -> IfVeSMSuStPassCmprtMd_Md29_CrtStat_Val/1
  ModeStatAndRsp_Runnable_sys/106(IfVeSMSuStPassCmprtMd_Md3_CrtStat_Val_write) -> IfVeSMSuStPassCmprtMd_Md3_CrtStat_Val/1
  ModeStatAndRsp_Runnable_sys/107(IfVeSMSuStPassCmprtMd_Md30_CrtStat_Val_write) -> IfVeSMSuStPassCmprtMd_Md30_CrtStat_Val/1
  ModeStatAndRsp_Runnable_sys/108(IfVeSMSuStPassCmprtMd_Md31_CrtStat_Val_write) -> IfVeSMSuStPassCmprtMd_Md31_CrtStat_Val/1
  ModeStatAndRsp_Runnable_sys/109(IfVeSMSuStPassCmprtMd_Md32_CrtStat_Val_write) -> IfVeSMSuStPassCmprtMd_Md32_CrtStat_Val/1
  ModeStatAndRsp_Runnable_sys/110(IfVeSMSuStPassCmprtMd_Md4_CrtStat_Val_write) -> IfVeSMSuStPassCmprtMd_Md4_CrtStat_Val/1
  ModeStatAndRsp_Runnable_sys/111(IfVeSMSuStPassCmprtMd_Md5_CrtStat_Val_write) -> IfVeSMSuStPassCmprtMd_Md5_CrtStat_Val/1
  ModeStatAndRsp_Runnable_sys/112(IfVeSMSuStPassCmprtMd_Md6_CrtStat_Val_write) -> IfVeSMSuStPassCmprtMd_Md6_CrtStat_Val/1
  ModeStatAndRsp_Runnable_sys/113(IfVeSMSuStPassCmprtMd_Md7_CrtStat_Val_write) -> IfVeSMSuStPassCmprtMd_Md7_CrtStat_Val/1
  ModeStatAndRsp_Runnable_sys/114(IfVeSMSuStPassCmprtMd_Md8_CrtStat_Val_write) -> IfVeSMSuStPassCmprtMd_Md8_CrtStat_Val/1
  ModeStatAndRsp_Runnable_sys/115(IfVeSMSuStPassCmprtMd_Md9_CrtStat_Val_write) -> IfVeSMSuStPassCmprtMd_Md9_CrtStat_Val/1
  ModeStatAndRsp_Runnable_sys/116(IfVeSMSuStPassCmprtMd10RclRspStat_Val_write) -> IfVeSMSuStPassCmprtMd10RclRspStat_Val/1
  ModeStatAndRsp_Runnable_sys/117(IfVeSMSuStPassCmprtMd11RclRspStat_Val_write) -> IfVeSMSuStPassCmprtMd11RclRspStat_Val/1
  ModeStatAndRsp_Runnable_sys/118(IfVeSMSuStPassCmprtMd12RclRspStat_Val_write) -> IfVeSMSuStPassCmprtMd12RclRspStat_Val/1
  ModeStatAndRsp_Runnable_sys/119(IfVeSMSuStPassCmprtMd13RclRspStat_Val_write) -> IfVeSMSuStPassCmprtMd13RclRspStat_Val/1
  ModeStatAndRsp_Runnable_sys/120(IfVeSMSuStPassCmprtMd14RclRspStat_Val_write) -> IfVeSMSuStPassCmprtMd14RclRspStat_Val/1
  ModeStatAndRsp_Runnable_sys/121(IfVeSMSuStPassCmprtMd15RclRspStat_Val_write) -> IfVeSMSuStPassCmprtMd15RclRspStat_Val/1
  ModeStatAndRsp_Runnable_sys/122(IfVeSMSuStPassCmprtMd16RclRspStat_Val_write) -> IfVeSMSuStPassCmprtMd16RclRspStat_Val/1
  ModeStatAndRsp_Runnable_sys/123(IfVeSMSuStPassCmprtMd17RclRspStat_Val_write) -> IfVeSMSuStPassCmprtMd17RclRspStat_Val/1
  ModeStatAndRsp_Runnable_sys/124(IfVeSMSuStPassCmprtMd18RclRspStat_Val_write) -> IfVeSMSuStPassCmprtMd18RclRspStat_Val/1
  ModeStatAndRsp_Runnable_sys/125(IfVeSMSuStPassCmprtMd19RclRspStat_Val_write) -> IfVeSMSuStPassCmprtMd19RclRspStat_Val/1
  ModeStatAndRsp_Runnable_sys/126(IfVeSMSuStPassCmprtMd1RclRspStat_Val_write) -> IfVeSMSuStPassCmprtMd1RclRspStat_Val/1
  ModeStatAndRsp_Runnable_sys/127(IfVeSMSuStPassCmprtMd20RclRspStat_Val_write) -> IfVeSMSuStPassCmprtMd20RclRspStat_Val/1
  ModeStatAndRsp_Runnable_sys/128(IfVeSMSuStPassCmprtMd21RclRspStat_Val_write) -> IfVeSMSuStPassCmprtMd21RclRspStat_Val/1
  ModeStatAndRsp_Runnable_sys/129(IfVeSMSuStPassCmprtMd22RclRspStat_Val_write) -> IfVeSMSuStPassCmprtMd22RclRspStat_Val/1
  ModeStatAndRsp_Runnable_sys/130(IfVeSMSuStPassCmprtMd23RclRspStat_Val_write) -> IfVeSMSuStPassCmprtMd23RclRspStat_Val/1
  ModeStatAndRsp_Runnable_sys/131(IfVeSMSuStPassCmprtMd24RclRspStat_Val_write) -> IfVeSMSuStPassCmprtMd24RclRspStat_Val/1
  ModeStatAndRsp_Runnable_sys/132(IfVeSMSuStPassCmprtMd25RclRspStat_Val_write) -> IfVeSMSuStPassCmprtMd25RclRspStat_Val/1
  ModeStatAndRsp_Runnable_sys/133(IfVeSMSuStPassCmprtMd26RclRspStat_Val_write) -> IfVeSMSuStPassCmprtMd26RclRspStat_Val/1
  ModeStatAndRsp_Runnable_sys/134(IfVeSMSuStPassCmprtMd27RclRspStat_Val_write) -> IfVeSMSuStPassCmprtMd27RclRspStat_Val/1
  ModeStatAndRsp_Runnable_sys/135(IfVeSMSuStPassCmprtMd28RclRspStat_Val_write) -> IfVeSMSuStPassCmprtMd28RclRspStat_Val/1
  ModeStatAndRsp_Runnable_sys/136(IfVeSMSuStPassCmprtMd29RclRspStat_Val_write) -> IfVeSMSuStPassCmprtMd29RclRspStat_Val/1
  ModeStatAndRsp_Runnable_sys/137(IfVeSMSuStPassCmprtMd2RclRspStat_Val_write) -> IfVeSMSuStPassCmprtMd2RclRspStat_Val/1
  ModeStatAndRsp_Runnable_sys/138(IfVeSMSuStPassCmprtMd30RclRspStat_Val_write) -> IfVeSMSuStPassCmprtMd30RclRspStat_Val/1
  ModeStatAndRsp_Runnable_sys/139(IfVeSMSuStPassCmprtMd31RclRspStat_Val_write) -> IfVeSMSuStPassCmprtMd31RclRspStat_Val/1
  ModeStatAndRsp_Runnable_sys/140(IfVeSMSuStPassCmprtMd32RclRspStat_Val_write) -> IfVeSMSuStPassCmprtMd32RclRspStat_Val/1
  ModeStatAndRsp_Runnable_sys/141(IfVeSMSuStPassCmprtMd3RclRspStat_Val_write) -> IfVeSMSuStPassCmprtMd3RclRspStat_Val/1
  ModeStatAndRsp_Runnable_sys/142(IfVeSMSuStPassCmprtMd4RclRspStat_Val_write) -> IfVeSMSuStPassCmprtMd4RclRspStat_Val/1
  ModeStatAndRsp_Runnable_sys/143(IfVeSMSuStPassCmprtMd5RclRspStat_Val_write) -> IfVeSMSuStPassCmprtMd5RclRspStat_Val/1
  ModeStatAndRsp_Runnable_sys/144(IfVeSMSuStPassCmprtMd6RclRspStat_Val_write) -> IfVeSMSuStPassCmprtMd6RclRspStat_Val/1
  ModeStatAndRsp_Runnable_sys/145(IfVeSMSuStPassCmprtMd7RclRspStat_Val_write) -> IfVeSMSuStPassCmprtMd7RclRspStat_Val/1
  ModeStatAndRsp_Runnable_sys/146(IfVeSMSuStPassCmprtMd8RclRspStat_Val_write) -> IfVeSMSuStPassCmprtMd8RclRspStat_Val/1
  ModeStatAndRsp_Runnable_sys/147(IfVeSMSuStPassCmprtMd9RclRspStat_Val_write) -> IfVeSMSuStPassCmprtMd9RclRspStat_Val/1
  ModeStatAndRsp_Runnable_sys/148(IfVeSMSuStSrv_StMd1_Rsp_Val_write) -> IfVeSMSuStSrv_StMd1_Rsp_Val/1
  ModeStatAndRsp_Runnable_sys/149(IfVeSMSuStSrv_StMd10_Rsp_Val_write) -> IfVeSMSuStSrv_StMd10_Rsp_Val/1
  ModeStatAndRsp_Runnable_sys/150(IfVeSMSuStSrv_StMd11_Rsp_Val_write) -> IfVeSMSuStSrv_StMd11_Rsp_Val/1
  ModeStatAndRsp_Runnable_sys/151(IfVeSMSuStSrv_StMd12_Rsp_Val_write) -> IfVeSMSuStSrv_StMd12_Rsp_Val/1
  ModeStatAndRsp_Runnable_sys/152(IfVeSMSuStSrv_StMd13_Rsp_Val_write) -> IfVeSMSuStSrv_StMd13_Rsp_Val/1
  ModeStatAndRsp_Runnable_sys/153(IfVeSMSuStSrv_StMd14_Rsp_Val_write) -> IfVeSMSuStSrv_StMd14_Rsp_Val/1
  ModeStatAndRsp_Runnable_sys/154(IfVeSMSuStSrv_StMd15_Rsp_Val_write) -> IfVeSMSuStSrv_StMd15_Rsp_Val/1
  ModeStatAndRsp_Runnable_sys/155(IfVeSMSuStSrv_StMd16_Rsp_Val_write) -> IfVeSMSuStSrv_StMd16_Rsp_Val/1
  ModeStatAndRsp_Runnable_sys/156(IfVeSMSuStSrv_StMd17_Rsp_Val_write) -> IfVeSMSuStSrv_StMd17_Rsp_Val/1
  ModeStatAndRsp_Runnable_sys/157(IfVeSMSuStSrv_StMd18_Rsp_Val_write) -> IfVeSMSuStSrv_StMd18_Rsp_Val/1
  ModeStatAndRsp_Runnable_sys/158(IfVeSMSuStSrv_StMd19_Rsp_Val_write) -> IfVeSMSuStSrv_StMd19_Rsp_Val/1
  ModeStatAndRsp_Runnable_sys/159(IfVeSMSuStSrv_StMd2_Rsp_Val_write) -> IfVeSMSuStSrv_StMd2_Rsp_Val/1
  ModeStatAndRsp_Runnable_sys/160(IfVeSMSuStSrv_StMd20_Rsp_Val_write) -> IfVeSMSuStSrv_StMd20_Rsp_Val/1
  ModeStatAndRsp_Runnable_sys/161(IfVeSMSuStSrv_StMd21_Rsp_Val_write) -> IfVeSMSuStSrv_StMd21_Rsp_Val/1
  ModeStatAndRsp_Runnable_sys/162(IfVeSMSuStSrv_StMd22_Rsp_Val_write) -> IfVeSMSuStSrv_StMd22_Rsp_Val/1
  ModeStatAndRsp_Runnable_sys/163(IfVeSMSuStSrv_StMd23_Rsp_Val_write) -> IfVeSMSuStSrv_StMd23_Rsp_Val/1
  ModeStatAndRsp_Runnable_sys/164(IfVeSMSuStSrv_StMd24_Rsp_Val_write) -> IfVeSMSuStSrv_StMd24_Rsp_Val/1
  ModeStatAndRsp_Runnable_sys/165(IfVeSMSuStSrv_StMd25_Rsp_Val_write) -> IfVeSMSuStSrv_StMd25_Rsp_Val/1
  ModeStatAndRsp_Runnable_sys/166(IfVeSMSuStSrv_StMd26_Rsp_Val_write) -> IfVeSMSuStSrv_StMd26_Rsp_Val/1
  ModeStatAndRsp_Runnable_sys/167(IfVeSMSuStSrv_StMd27_Rsp_Val_write) -> IfVeSMSuStSrv_StMd27_Rsp_Val/1
  ModeStatAndRsp_Runnable_sys/168(IfVeSMSuStSrv_StMd28_Rsp_Val_write) -> IfVeSMSuStSrv_StMd28_Rsp_Val/1
  ModeStatAndRsp_Runnable_sys/169(IfVeSMSuStSrv_StMd29_Rsp_Val_write) -> IfVeSMSuStSrv_StMd29_Rsp_Val/1
  ModeStatAndRsp_Runnable_sys/170(IfVeSMSuStSrv_StMd3_Rsp_Val_write) -> IfVeSMSuStSrv_StMd3_Rsp_Val/1
  ModeStatAndRsp_Runnable_sys/171(IfVeSMSuStSrv_StMd30_Rsp_Val_write) -> IfVeSMSuStSrv_StMd30_Rsp_Val/1
  ModeStatAndRsp_Runnable_sys/172(IfVeSMSuStSrv_StMd31_Rsp_Val_write) -> IfVeSMSuStSrv_StMd31_Rsp_Val/1
  ModeStatAndRsp_Runnable_sys/173(IfVeSMSuStSrv_StMd32_Rsp_Val_write) -> IfVeSMSuStSrv_StMd32_Rsp_Val/1
  ModeStatAndRsp_Runnable_sys/174(IfVeSMSuStSrv_StMd4_Rsp_Val_write) -> IfVeSMSuStSrv_StMd4_Rsp_Val/1
  ModeStatAndRsp_Runnable_sys/175(IfVeSMSuStSrv_StMd5_Rsp_Val_write) -> IfVeSMSuStSrv_StMd5_Rsp_Val/1
  ModeStatAndRsp_Runnable_sys/176(IfVeSMSuStSrv_StMd6_Rsp_Val_write) -> IfVeSMSuStSrv_StMd6_Rsp_Val/1
  ModeStatAndRsp_Runnable_sys/177(IfVeSMSuStSrv_StMd7_Rsp_Val_write) -> IfVeSMSuStSrv_StMd7_Rsp_Val/1
  ModeStatAndRsp_Runnable_sys/178(IfVeSMSuStSrv_StMd8_Rsp_Val_write) -> IfVeSMSuStSrv_StMd8_Rsp_Val/1
  ModeStatAndRsp_Runnable_sys/179(IfVeSMSuStSrv_StMd9_Rsp_Val_write) -> IfVeSMSuStSrv_StMd9_Rsp_Val/1
  INTMMdReq_Val/1 -> ModeStatAndRsp_Runnable_sys/83(INTMMdReq_Val_read)
  INTMSrcReqTp_Val/1 -> ModeStatAndRsp_Runnable_sys/84(INTMSrcReqTp_Val_read)
  LfFamlyReq_Val/1 -> ModeStatAndRsp_Runnable_sys/85(LfFamlyReq_Val_read)
  LfFamlySrcReqTp_Val/1 -> ModeStatAndRsp_Runnable_sys/86(LfFamlySrcReqTp_Val_read)
  LfLyMdReq_Val/1 -> ModeStatAndRsp_Runnable_sys/87(LfLyMdReq_Val_read)
  LfLySrcReqTp_Val/1 -> ModeStatAndRsp_Runnable_sys/88(LfLySrcReqTp_Val_read)
  RtFamlyMdReq_Val/1 -> ModeStatAndRsp_Runnable_sys/89(RtFamlyMdReq_Val_read)
  RtFamlySrcReqTp_Val/1 -> ModeStatAndRsp_Runnable_sys/90(RtFamlySrcReqTp_Val_read)
  RtLyMdReq_Val/1 -> ModeStatAndRsp_Runnable_sys/91(RtLyMdReq_Val_read)
  RtLySrcReqTp_Val/1 -> ModeStatAndRsp_Runnable_sys/92(RtLySrcReqTp_Val_read)
  SoftIntINTM_Val/1 -> ModeStatAndRsp_Runnable_sys/93(SoftIntINTM_Val_read)
  SoftIntLfFamly_Val/1 -> ModeStatAndRsp_Runnable_sys/94(SoftIntLfFamly_Val_read)
  SoftIntLfLy_Val/1 -> ModeStatAndRsp_Runnable_sys/95(SoftIntLfLy_Val_read)
  SoftIntRtFamly_Val/1 -> ModeStatAndRsp_Runnable_sys/96(SoftIntRtFamly_Val_read)
  SoftIntRtLy_Val/1 -> ModeStatAndRsp_Runnable_sys/97(SoftIntRtLy_Val_read)
  SwIntINTM_Val/1 -> ModeStatAndRsp_Runnable_sys/98(SwIntINTM_Val_read)
  SwIntLfFamly_Val/1 -> ModeStatAndRsp_Runnable_sys/99(SwIntLfFamly_Val_read)
  SwIntLfLy_Val/1 -> ModeStatAndRsp_Runnable_sys/100(SwIntLfLy_Val_read)
  SwIntRtFamly_Val/1 -> ModeStatAndRsp_Runnable_sys/101(SwIntRtFamly_Val_read)
  SwIntRtLy_Val/1 -> ModeStatAndRsp_Runnable_sys/102(SwIntRtLy_Val_read)
  PosArray_Val/1 -> ModeStatAndRsp_Runnable_sys/103(PosArray_Val_read)
  AllVipSrcReqTp_Val/1 -> ModeStatAndRsp_Runnable_sys/104(AllVipSrcReqTp_Val_read)
  LugMdLtAvl_Val/1 -> ModeStatAndRsp_Runnable_sys/105(LugMdLtAvl_Val_read)
  LugMdRtAvl_Val/1 -> ModeStatAndRsp_Runnable_sys/106(LugMdRtAvl_Val_read)
  VipMdLtAvl_Val/1 -> ModeStatAndRsp_Runnable_sys/107(VipMdLtAvl_Val_read)
  VipMdRtAvl_Val/1 -> ModeStatAndRsp_Runnable_sys/108(VipMdRtAvl_Val_read)
  SwIntAllVip_Val/1 -> ModeStatAndRsp_Runnable_sys/109(SwIntAllVip_Val_read)
  IfVeSMSeStNumConfig_Val/1 -> ModeStatAndRsp_Runnable_sys/110(IfVeSMSeStNumConfig_Val_read)
  IntimacyRtMdReq_Val/1 -> ModeStatAndRsp_Runnable_sys/111(IntimacyRtMdReq_Val_read)
  IntimacyRtMdSrcTp_Val/1 -> ModeStatAndRsp_Runnable_sys/112(IntimacyRtMdSrcTp_Val_read)
  isINTMRArrivedAtTargetPos_Val/1 -> ModeStatAndRsp_Runnable_sys/113(isINTMRArrivedAtTargetPos_Val_read)
  isINTMRDoneFailed_Val/1 -> ModeStatAndRsp_Runnable_sys/114(isINTMRDoneFailed_Val_read)
  isINTMRDoneOK_Val/1 -> ModeStatAndRsp_Runnable_sys/115(isINTMRDoneOK_Val_read)
  isLgrstCloseLArrivedAtTargetPos_Val/1 -> ModeStatAndRsp_Runnable_sys/116(isLgrstCloseLArrivedAtTargetPos_Val_read)
  isLgrstCloseLDoneFailed_Val/1 -> ModeStatAndRsp_Runnable_sys/117(isLgrstCloseLDoneFailed_Val_read)
  isLgrstCloseLDoneOK_Val/1 -> ModeStatAndRsp_Runnable_sys/118(isLgrstCloseLDoneOK_Val_read)
  isLgrstCloseRArrivedAtTargetPos_Val/1 -> ModeStatAndRsp_Runnable_sys/119(isLgrstCloseRArrivedAtTargetPos_Val_read)
  isLgrstCloseRDoneFailed_Val/1 -> ModeStatAndRsp_Runnable_sys/120(isLgrstCloseRDoneFailed_Val_read)
  isLgrstCloseRDoneOK_Val/1 -> ModeStatAndRsp_Runnable_sys/121(isLgrstCloseRDoneOK_Val_read)
  isLgrstOpenLArrivedAtTargetPos_Val/1 -> ModeStatAndRsp_Runnable_sys/122(isLgrstOpenLArrivedAtTargetPos_Val_read)
  isLgrstOpenLDoneFailed_Val/1 -> ModeStatAndRsp_Runnable_sys/123(isLgrstOpenLDoneFailed_Val_read)
  isLgrstOpenLDoneOK_Val/1 -> ModeStatAndRsp_Runnable_sys/124(isLgrstOpenLDoneOK_Val_read)
  isLgrstOpenRArrivedAtTargetPos_Val/1 -> ModeStatAndRsp_Runnable_sys/125(isLgrstOpenRArrivedAtTargetPos_Val_read)
  isLgrstOpenRDoneFailed_Val/1 -> ModeStatAndRsp_Runnable_sys/126(isLgrstOpenRDoneFailed_Val_read)
  isLgrstOpenRDoneOK_Val/1 -> ModeStatAndRsp_Runnable_sys/127(isLgrstOpenRDoneOK_Val_read)
  LgrstCloseLtMdReq_Val/1 -> ModeStatAndRsp_Runnable_sys/128(LgrstCloseLtMdReq_Val_read)
  LgrstCloseLtSrcReqTp_Val/1 -> ModeStatAndRsp_Runnable_sys/129(LgrstCloseLtSrcReqTp_Val_read)
  LgrstCloseRtMdReq_Val/1 -> ModeStatAndRsp_Runnable_sys/130(LgrstCloseRtMdReq_Val_read)
  LgrstCloseRtSrcReqTp_Val/1 -> ModeStatAndRsp_Runnable_sys/131(LgrstCloseRtSrcReqTp_Val_read)
  LgrstOpenLtMdReq_Val/1 -> ModeStatAndRsp_Runnable_sys/132(LgrstOpenLtMdReq_Val_read)
  LgrstOpenLtSrcReqTp_Val/1 -> ModeStatAndRsp_Runnable_sys/133(LgrstOpenLtSrcReqTp_Val_read)
  LgrstOpenRtMdReq_Val/1 -> ModeStatAndRsp_Runnable_sys/134(LgrstOpenRtMdReq_Val_read)
  LgrstOpenRtSrcReqTp_Val/1 -> ModeStatAndRsp_Runnable_sys/135(LgrstOpenRtSrcReqTp_Val_read)
  SoftIntIntimacyRt_Val/1 -> ModeStatAndRsp_Runnable_sys/136(SoftIntIntimacyRt_Val_read)
  SoftIntLgrstCloseLt_Val/1 -> ModeStatAndRsp_Runnable_sys/137(SoftIntLgrstCloseLt_Val_read)
  SoftIntLgrstCloseRt_Val/1 -> ModeStatAndRsp_Runnable_sys/138(SoftIntLgrstCloseRt_Val_read)
  SoftIntLgrstOpenLt_Val/1 -> ModeStatAndRsp_Runnable_sys/139(SoftIntLgrstOpenLt_Val_read)
  SoftIntLgrstOpenRt_Val/1 -> ModeStatAndRsp_Runnable_sys/140(SoftIntLgrstOpenRt_Val_read)
  SwIntIntimacyRt_Val/1 -> ModeStatAndRsp_Runnable_sys/141(SwIntIntimacyRt_Val_read)
  SwIntLgrstCloseLt_Val/1 -> ModeStatAndRsp_Runnable_sys/142(SwIntLgrstCloseLt_Val_read)
  SwIntLgrstCloseRt_Val/1 -> ModeStatAndRsp_Runnable_sys/143(SwIntLgrstCloseRt_Val_read)
  SwIntLgrstOpenLt_Val/1 -> ModeStatAndRsp_Runnable_sys/144(SwIntLgrstOpenLt_Val_read)
  SwIntLgrstOpenRt_Val/1 -> ModeStatAndRsp_Runnable_sys/145(SwIntLgrstOpenRt_Val_read)
